simulink model "WSCC_Indian_400kV"  (R2022a)
settings: Solver=FixedStepDiscrete  StartTime=0.0  StopTime=1  FixedStep=5e-7  RelTol=1e-3
PreLoadFcn:
  | tf=1e-3
  | to=20e-3
model workspace (MAT data in the model file):
  tf = 0.001
  to = 0.02
undefined symbols (not defined in the file or in its folder): D1, Delta
libraries: spsFourierLib x72, spsThreePhaseVIMeasurementLib x21, spsThreePhaseBreakerLib x12, spsDistributedParametersLineLib x12, spsLoadFlowBusLib x9, spsThreePhaseParallelRLCLoadLib x6, spsThreePhaseSeriesRLCLoadLib x3, spsThreePhaseSourceLib x3, spsThreePhaseTransformerTwoWindingsLib x3, spsThreePhaseFaultLib x1, spspowerguiLib x1
(part 1 of 2)
settings Model: ParameterArgumentNames=tf,to  Creator=MARI  LastModifiedBy=Dell
settings SolverCC: AlgebraicLoopSolver=TrustRegion
settings DataIOCC: SignalLogging=off  DSMLogging=off
settings DebuggingCC: SFMachineParentedDataDiag=warning  ArithmeticOperatorsInVariantConditions=warning
settings SFSimCC: SimUseLocalCustomCode=off  CustomCodeUndefinedFunction=UseInterfaceOnly
settings RTWCC: RTWUseLocalCustomCode=off  DLArmComputeVersion=19.05

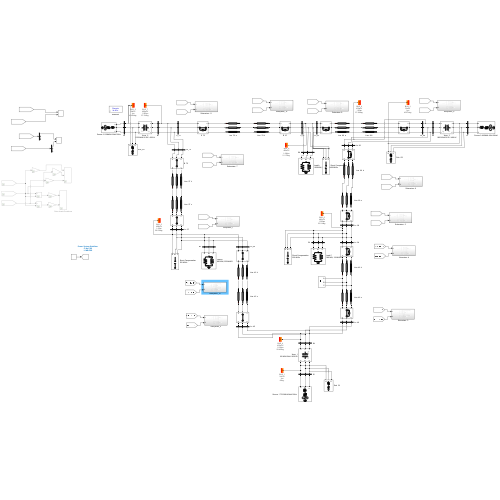
[thumbnail: Simulink's stored preview of the top-level diagram]
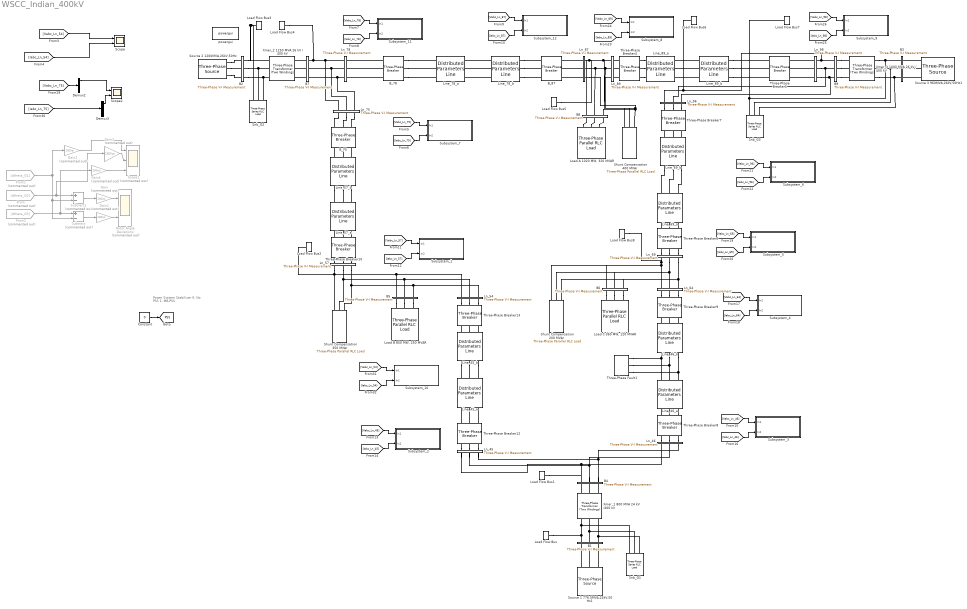
== system WSCC_Indian_400kV ==
  note: Power System Stabilizer
      | 0: No PSS
      | 1: MB-PSS
  B1 : spsThreePhaseVIMeasurementLib/Three-Phase V-I Measurement  VoltageMeasurement=phase-to-ground  SetLabelV=on  LabelV=Vabc_G1  Vpu=off  VpuLL=off  CurrentMeasurement=yes  SetLabelI=on  LabelI=Iabc_G1  Ipu=off  Pbase=100e6  Vbase=500e3  OutputType=Complex  PhasorSimulation=off  PSBequivalent=0
  B2 : spsThreePhaseVIMeasurementLib/Three-Phase V-I Measurement  VoltageMeasurement=phase-to-ground  SetLabelV=on  LabelV=Vabc_G2  Vpu=off  VpuLL=off  CurrentMeasurement=yes  SetLabelI=on  LabelI=Iabc_G2  Ipu=off  Pbase=100e6  Vbase=500e3  OutputType=Complex  PhasorSimulation=off  PSBequivalent=0
  B3 : spsThreePhaseVIMeasurementLib/Three-Phase V-I Measurement  VoltageMeasurement=phase-to-ground  SetLabelV=on  LabelV=Vabc_G3  Vpu=off  VpuLL=off  CurrentMeasurement=yes  SetLabelI=on  LabelI=Iabc_G3  Ipu=off  Pbase=100e6  Vbase=500e3  OutputType=Complex  PhasorSimulation=off  PSBequivalent=0
  B4 : spsThreePhaseVIMeasurementLib/Three-Phase V-I Measurement  VoltageMeasurement=phase-to-ground  SetLabelV=on  LabelV=Vabc_X1  Vpu=off  VpuLL=off  CurrentMeasurement=yes  SetLabelI=on  LabelI=Iabc_X1  Ipu=off  Pbase=100e6  Vbase=500e3  OutputType=Complex  PhasorSimulation=off  PSBequivalent=0
  B5 : spsThreePhaseVIMeasurementLib/Three-Phase V-I Measurement  VoltageMeasurement=phase-to-ground  SetLabelV=on  LabelV=Vabc_Ld_B  Vpu=off  VpuLL=off  CurrentMeasurement=yes  SetLabelI=on  LabelI=Iabc_Ld_B  Ipu=off  Pbase=100e6  Vbase=500e3  OutputType=Complex  PhasorSimulation=off  PSBequivalent=0
  B6 : spsThreePhaseVIMeasurementLib/Three-Phase V-I Measurement  VoltageMeasurement=phase-to-ground  SetLabelV=on  LabelV=Vabc_Ld_C  Vpu=off  VpuLL=off  CurrentMeasurement=yes  SetLabelI=on  LabelI=Iabc_Ld_C  Ipu=off  Pbase=100e6  Vbase=500e3  OutputType=Complex  PhasorSimulation=off  PSBequivalent=0
  B7 : spsThreePhaseVIMeasurementLib/Three-Phase V-I Measurement  VoltageMeasurement=phase-to-ground  SetLabelV=on  LabelV=Vabc_X2  Vpu=off  VpuLL=off  CurrentMeasurement=yes  SetLabelI=on  LabelI=Iabc_X2  Ipu=off  Pbase=100e6  Vbase=500e3  OutputType=Complex  PhasorSimulation=off  PSBequivalent=0
  B8 : spsThreePhaseVIMeasurementLib/Three-Phase V-I Measurement  VoltageMeasurement=phase-to-ground  SetLabelV=on  LabelV=Vabc_Ld_A  Vpu=off  VpuLL=off  CurrentMeasurement=yes  SetLabelI=on  LabelI=Iabc_Ld_A  Ipu=off  Pbase=100e6  Vbase=500e3  OutputType=Complex  PhasorSimulation=off  PSBequivalent=0
  B9 : spsThreePhaseVIMeasurementLib/Three-Phase V-I Measurement  VoltageMeasurement=phase-to-ground  SetLabelV=on  LabelV=Vabc_X3  Vpu=off  VpuLL=off  CurrentMeasurement=yes  SetLabelI=on  LabelI=Iabc_X3  Ipu=off  Pbase=100e6  Vbase=500e3  OutputType=Complex  PhasorSimulation=off  PSBequivalent=0
  B_75 : spsThreePhaseBreakerLib/Three-Phase Breaker  InitialState=closed  SwitchA=on  SwitchB=on  SwitchC=on  SwitchTimes=[500 501]  External=off  BreakerResistance=0.01  SnubberResistance=inf  SnubberCapacitance=inf  Measurements=None
  B_78 : spsThreePhaseBreakerLib/Three-Phase Breaker  InitialState=closed  SwitchA=on  SwitchB=on  SwitchC=on  SwitchTimes=[500 501]  External=off  BreakerResistance=0.01  SnubberResistance=10e6  SnubberCapacitance=inf  Measurements=None
  B_87 : spsThreePhaseBreakerLib/Three-Phase Breaker  InitialState=closed  SwitchA=on  SwitchB=on  SwitchC=on  SwitchTimes=[500 501]  External=off  BreakerResistance=0.01  SnubberResistance=10e6  SnubberCapacitance=inf  Measurements=None
  Constant : Constant  Value=0
  Demux2 : Demux  Outputs=3
  Demux3 : Demux  Outputs=3
  From : From  Commented=on  GotoTag=dtheta_G2
  From1 : From  Commented=on  GotoTag=dtheta_G1
  From2 : From  Commented=on  GotoTag=dtheta_G3
  Gain{,1..4} (5 alike) : Gain  Commented=on  Gain=180/pi
  Line_45_a : spsDistributedParametersLineLib/Distributed Parameters Line  Phases=3  Length=90  Frequency=50  Resistance=[0.0298 0.1619]  Inductance=[1.0568e-03 3.9470e-03]  Capacitance=[11.0414e-09 7.1301e-09]  x1=[-0.00048 -0.000500323391905853 302835.955606375 -284216.33245044;-0.00046 -0.000500693757200361 304615.750015299 -282307.960357671;-0.00044 -0.00050104435596266 306383.518715997 -280388.443230016;-0.00042 -0.00050137517435171 308139.19191999 -278457.856846725;-0.0004 -0.000501686199307369 309882.700316304 -276516.277424041;-0.00038 -0.000501977418550903 311613.975074215 -274563.781612196;-0.00036 -0.000502248820585476 313332.947845957 -272600.446492382;-0.00034 -0.000502500394696601 315039.550769431 -270626.349573707;-0.00032 -0.000502732130952561 316733.716470874 -268641.568790137;-0.0003 -0.000502944020204806 318415.378067527 -266646.18249742;-0.00028 -0.000503136054088312 320084.469170267 -264640.269469989;-0.00026 -0.000503308225021909 321740.923886237 -262623.908897855;-0.00024 -0.000503460526208584 323384.676821441 -260597.180383483;-0.00022 -0.000503592951635747 325015.663083327 -258560.163938643;-0.0002 -0.000503705496075468 326633.818283351 -256512.939981257;-0.00018 -0.000503798155084687 328239.078539515 -254455.589332221;-0.00016 -0.000503870925005383 329831.380478894 -252388.193212216;-0.00014 -0.000503923802964725 331410.661240133 -250310.8332385;-0.00012 -0.000503956786875182 332976.858475933 -248223.591421689;-0.0001 -0.000503969875434606 334529.910355508 -246126.550162516;-8e-05 -0.000503963068126281 336069.755567029 -244019.792248578;-6e-05 -0.000503936365218951 337596.333320043 -241903.400851071;-4e-05 -0.000503889767766798 339109.583347876 -239777.459521504;-2e-05 -0.000503823277609412 340609.445910006 -237642.052188399]  x2=[-0.00048 -0.000256541905604458 288659.111644199 -303840.350628517;-0.00046 -0.000258441737311412 290562.486422962 -302020.666326207;-0.00044 -0.0002603313661811 292454.390292283 -300189.058765133;-0.00042 -0.000262210717614209 294334.748563038 -298345.600254026;-0.0004 -0.000264079717417164 296203.487001901 -296490.363569469;-0.00038 -0.000265938291805053 298060.53183428 -294623.421953032;-0.00036 -0.00026778636740454 299905.809747222 -292744.849108372;-0.00034 -0.000269623871256766 301739.247892317 -290854.719198329;-0.00032 -0.000271450730820224 303560.773888566 -288953.106841995;-0.0003 -0.000273266873973628 305370.315825241 -287040.087111769;-0.00028 -0.000275072229018755 307167.802264724 -285115.735530396;-0.00026 -0.00027686672468328 308953.16224533 -283180.128067981;-0.00024 -0.000278650290123586 310726.325284103 -281233.341138991;-0.00022 -0.000280422854927563 312487.221379602 -279275.451599242;-0.0002 -0.000282184349117389 314235.781014665 -277306.53674286;-0.00018 -0.000283934703152289 315971.935159152 -275326.674299232;-0.00016 -0.000285673847931282 317695.615272669 -273335.942429938;-0.00014 -0.000287401714795911 319406.753307277 -271334.419725662;-0.00012 -0.00028911823553295 321105.281710177 -269322.185203095;-0.0001 -0.0002908233423771 322791.133426374 -267299.318301809;-8e-05 -0.000292516968013663 324464.241901332 -265265.898881127;-6e-05 -0.000294199045581198 326124.54108359 -263222.007216964;-4e-05 -0.000295869508674162 327771.965427381 -261167.723998665;-2e-05 -0.000297528291345534 329406.449895213 -259103.130325814]  x3=[-0.00048 1.74609434734278e-06 236.557476392391 -548.665991316306;-0.00046 1.75692178428303e-06 240.00015435941 -547.16883645487;-0.00044 1.76767986095957e-06 243.433357531282 -545.650080304675;-0.00042 1.77836815266196e-06 246.856950371023 -544.109782823612;-0.0004 1.78898623743472e-06 250.27079772105 -542.548004819988;-0.00038 1.79953369609407e-06 253.674764808515 -540.964807950125;-0.00036 1.8100101122444e-06 257.068717250626 -539.360254715924;-0.00034 1.82041507229472e-06 260.452521059953 -537.7344084624;-0.00032 1.83074816547504e-06 263.826042649714 -536.087333375178;-0.0003 1.84100898385253e-06 267.189148839054 -534.419094477964;-0.00028 1.85119712234765e-06 270.541706858299 -532.729757629971;-0.00026 1.86131217875014e-06 273.883584354198 -531.019389523326;-0.00024 1.87135375373489e-06 277.214649395152 -529.288057680434;-0.00022 1.88132145087771e-06 280.534770476414 -527.535830451311;-0.0002 1.89121487667099e-06 283.843816525291 -525.762777010888;-0.00018 1.90103364053922e-06 287.141656906309 -523.968967356279;-0.00016 1.9107773548544e-06 290.428161426379 -522.154472304017;-0.00014 1.9204456349514e-06 293.703200339928 -520.319363487259;-0.00012 1.93003809914305e-06 296.966644354027 -518.463713352961;-0.0001 1.93955436873531e-06 300.218364633496 -516.587595159012;-8e-05 1.94899406804214e-06 303.458232805986 -514.691082971346;-6e-05 1.95835682440037e-06 306.686120967048 -512.774251661016;-4e-05 1.96764226818442e-06 309.901901685185 -510.837176901241;-2e-05 1.97685003282087e-06 313.105448006881 -508.879935164415]  x4=[-0.00048 -2.71213831700393e-06 1571.48762055538 -1431.8045403172;-0.00046 -2.72644875026853e-06 1580.45283477776 -1421.90239475558;-0.00044 -2.7406515480049e-06 1589.35565542839 -1411.9441149221;-0.00042 -2.75474614951091e-06 1598.19573103915 -1401.93009395259;-0.0004 -2.76873199835581e-06 1606.97271261901 -1391.86072718347;-0.00038 -2.78260854240224e-06 1615.68625366775 -1381.73641213608;-0.00036 -2.79637523382801e-06 1624.33601018969 -1371.55754850106;-0.00034 -2.81003152914771e-06 1632.92164070726 -1361.3245381225;-0.00032 -2.82357688923419e-06 1641.44280627446 -1351.03778498214;-0.0003 -2.83701077933981e-06 1649.89917049027 -1340.69769518337;-0.00028 -2.85033266911761e-06 1658.29039951191 -1330.30467693524;-0.00026 -2.86354203264218e-06 1666.61616206803 -1319.85914053631;-0.00024 -2.87663834843047e-06 1674.87612947177 -1309.36149835848;-0.00022 -2.88962109946236e-06 1683.06997563377 -1298.81216483067;-0.0002 -2.90248977320107e-06 1691.19737707501 -1288.21155642252;-0.00018 -2.91524386161339e-06 1699.25801293959 -1277.56009162789;-0.00016 -2.92788286118975e-06 1707.25156500742 -1266.85819094838;-0.00014 -2.94040627296409e-06 1715.17771770674 -1256.1062768767;-0.00012 -2.95281360253355e-06 1723.03615812663 -1245.30477388001;-0.0001 -2.96510436007801e-06 1730.8265760293 -1234.45410838315;-8e-05 -2.97727806037941e-06 1738.5486638624 -1223.55470875181;-6e-05 -2.9893342228409e-06 1746.20211677112 -1212.60700527563;-4e-05 -3.00127237150584e-06 1753.78663261025 -1201.6114301512;-2e-05 -3.01309203507655e-06 1761.30191195609 -1190.568417465]  x5=0.00047744558650175  V1=[1.62e-10 4.153e+05 4.153e+05;314.2 314.2 314.2;-0.6943 0.8874 -0.6834]  V2=[8.471e-10 4.186e+05 4.186e+05;314.2 314.2 314.2;-0.039 0.8395 -0.7313]  I1=[7.601e-12 598 598;314.2 314.2 314.2;-1.312 0.4775 -1.093]  I2=[4.421e-12 2129 2129;314.2 314.2 314.2;2.105 0.9183 -0.6525]  nHarmo=1  Measurements=None  Decoupling=off  VsMag0=0  VrMag0=0  VsAngle0=0  VrAngle0=0  IsMag0=0  IrMag0=0  IsAngle0=0  IrAngle0=0
      settings: SourceProductBaseCode=PS
  Line_45_b : spsDistributedParametersLineLib/Distributed Parameters Line  Phases=3  Length=60  Frequency=50  Resistance=[0.0298 0.1619]  Inductance=[1.0568e-03 3.9470e-03]  Capacitance=[11.0414e-09 7.1301e-09]  x1=[-0.00032 -0.000271450732280679 303560.773888566 -288953.106841995;-0.0003 -0.000273266875343084 305370.315825241 -287040.087111769;-0.00028 -0.000275072230297158 307167.802264724 -285115.735530396;-0.00026 -0.000276866725870579 308953.16224533 -283180.128067981;-0.00024 -0.000278650291219735 310726.325284103 -281233.341138991;-0.00022 -0.000280422855932519 312487.221379602 -279275.451599242;-0.0002 -0.000282184350031111 314235.781014665 -277306.53674286;-0.00018 -0.000283934703974742 315971.935159152 -275326.674299232;-0.00016 -0.000285673848662433 317695.615272669 -273335.942429938;-0.00014 -0.000287401715435731 319406.753307277 -271334.419725662;-0.00012 -0.000289118236081415 321105.281710177 -269322.185203095;-0.0001 -0.000290823342834187 322791.133426374 -267299.318301809;-8e-05 -0.000292516968379354 324464.241901332 -265265.898881127;-6e-05 -0.000294199045855478 326124.54108359 -263222.007216964;-4e-05 -0.000295869508857022 327771.965427381 -261167.723998665;-2e-05 -0.000297528291436966 329406.449895213 -259103.130325814]  x2=[-0.00032 -0.000113963482428579 293331.273337558 -300866.465593188;-0.0003 -0.000116825548862926 295215.870543759 -299017.484128223;-0.00028 -0.000119683003224641 297088.813132882 -297156.697964984;-0.00026 -0.000122535732706319 298950.02716436 -295284.180564123;-0.00024 -0.000125383624687085 300799.43916065 -293400.005849421;-0.00022 -0.000128226566737039 302636.976110133 -291504.24820487;-0.0002 -0.000131064446621698 304462.565469997 -289596.982471735;-0.00018 -0.000133897152306422 306276.1351691 -287678.283945601;-0.00016 -0.000136724571960841 308077.613610815 -285748.228373401;-0.00014 -0.00013954659396327 309866.929675857 -283806.891950424;-0.00012 -0.000142363106905111 311644.012725094 -281854.351317308;-0.0001 -0.000145173999595256 313408.792602328 -279890.683557014;-8e-05 -0.000147979161064475 315161.199637071 -277915.966191783;-6e-05 -0.000150778480569796 316901.164647296 -275930.277180075;-4e-05 -0.000153571847598878 318628.618942162 -273933.694913492;-2e-05 -0.000156359151874374 320343.494324732 -271926.298213684]  x3=[-0.00032 2.11081364469373e-06 309.410896766023 -506.244452632187;-0.0003 2.11946097416425e-06 312.58559603185 -504.290386606476;-0.00028 2.12802463094461e-06 315.747954953577 -502.316412059784;-0.00026 2.13650427695629e-06 318.89784868669 -500.322606921248;-0.00024 2.14489957743741e-06 322.035152878777 -498.30904990288;-0.00022 2.15321020095586e-06 325.159743674441 -496.275820496463;-0.0002 2.16143581942247e-06 328.271497720188 -494.222998970414;-0.00018 2.1695761081039e-06 331.370292169295 -492.15066636661;-0.00016 2.17763074563549e-06 334.456004686665 -490.058904497196;-0.00014 2.18559941403394e-06 337.528513453649 -487.947795941347;-0.00012 2.19348179870987e-06 340.587697172864 -485.817424042015;-0.0001 2.20127758848023e-06 343.633435072975 -483.667872902634;-8e-05 2.20898647558059e-06 346.665606913463 -481.499227383803;-6e-05 2.21660815567728e-06 349.684092989376 -479.311573099934;-4e-05 2.22414232787943e-06 352.688774136054 -477.104996415872;-2e-05 2.23158869475082e-06 355.679531733829 -474.879584443485]  x4=[-0.00032 -2.57395052999193e-06 1550.37311665751 -1453.95656083358;-0.0003 -2.58898708897482e-06 1559.47793199607 -1444.18664347805;-0.00028 -2.60392143918049e-06 1568.52118181613 -1434.35971210668;-0.00026 -2.61875299102637e-06 1577.50250910567 -1424.4761546699;-0.00024 -2.63348115898819e-06 1586.42155929727 -1414.53636135362;-0.00022 -2.64810536162309e-06 1595.27798028209 -1404.54072456387;-0.0002 -2.66262502159259e-06 1604.07142242381 -1394.48963891127;-0.00018 -2.67703956568539e-06 1612.80153857238 -1384.38350119548;-0.00016 -2.69134842483997e-06 1621.46798407777 -1374.22271038951;-0.00014 -2.70555103416705e-06 1630.07041680354 -1364.00766762397;-0.00012 -2.71964683297195e-06 1638.60849714038 -1353.73877617127;-0.0001 -2.73363526477667e-06 1647.08188801951 -1343.41644142966;-8e-05 -2.74751577734187e-06 1655.49025492595 -1333.04107090725;-6e-05 -2.76128782268868e-06 1663.83326591178 -1322.61307420588;-4e-05 -2.77495085712033e-06 1672.11059160921 -1312.13286300502;-2e-05 -2.78850434124362e-06 1680.3219052436 -1301.60085104546]  x5=0.000318297057667833  V1=[8.377e-10 4.186e+05 4.186e+05;314.2 314.2 314.2;-0.02057 0.8395 -0.7313]  V2=[8.866e-10 4.202e+05 4.202e+05;314.2 314.2 314.2;-0.5299 0.7927 -0.7781]  I1=[5.663e-12 593.1 593.1;314.2 314.2 314.2;-2.774 0.5529 -1.018]  I2=[8.582e-12 2124 2124;314.2 314.2 314.2;-0.07241 0.8375 -0.7333]  nHarmo=1  Measurements=None  Decoupling=off  VsMag0=0  VrMag0=0  VsAngle0=0  VrAngle0=0  IsMag0=0  IrMag0=0  IsAngle0=0  IrAngle0=0
      settings: SourceProductBaseCode=PS
  Line_46_a : spsDistributedParametersLineLib/Distributed Parameters Line  Phases=3  Length=60  Frequency=50  Resistance=[0.0298 0.1619]  Inductance=[1.0568e-03 3.9470e-03]  Capacitance=[11.0414e-09 7.1301e-09]  x1=[-0.00032 -0.000503298405632093 316737.218945027 -268645.514115454;-0.0003 -0.000503514299837074 318418.905261583 -266650.105738309;-0.00028 -0.000503710316159651 320088.02094498 -264644.170471566;-0.00026 -0.000503886446861437 321744.500101388 -262627.787506117;-0.00024 -0.000504042684989092 323388.277335847 -260601.036445308;-0.00022 -0.000504179024374603 325019.287754846 -258563.997301801;-0.0002 -0.000504295459635525 326637.466968887 -256516.750494413;-0.00018 -0.000504391986175192 328242.751095025 -254459.376844942;-0.00016 -0.000504468600182903 329835.076759391 -252391.957574977;-0.00014 -0.000504525298634067 331414.381099695 -250314.574302692;-0.00012 -0.000504562079290327 332980.601767706 -248227.30903962;-0.0001 -0.000504578940699645 334533.676931713 -246130.244187421;-8e-05 -0.000504575882196361 336073.545278968 -244023.462534624;-6e-05 -0.000504552903901221 337600.146018105 -241907.047253361;-4e-05 -0.000504510006721368 339113.418881542 -239781.081896084;-2e-05 -0.000504447192350309 340613.304127856 -237645.650392264]  x2=[-0.00032 -0.000448622268654471 316728.936456653 -276237.738045629;-0.0003 -0.000449366397899025 318458.325972699 -274242.231844579;-0.00028 -0.000450092786927629 320175.143299322 -272235.899029795;-0.00026 -0.000450801407063687 321879.320659516 -270218.818807859;-0.00024 -0.000451492230332091 323570.790775277 -268191.070809645;-0.00022 -0.000452165229460319 325249.486870259 -266152.735087172;-0.0002 -0.000452820377879519 326915.342672416 -264103.892110445;-0.00018 -0.000453457649725553 328568.292416613 -262044.622764275;-0.00016 -0.000454077019840019 330208.270847224 -259975.008345091;-0.00014 -0.000454678463771247 331835.21322071 -257895.130557726;-0.00012 -0.000455261957775259 333449.05530817 -255805.071512194;-0.0001 -0.000455827478816712 335049.733397883 -253704.913720447;-8e-05 -0.000456375004569803 336637.184297819 -251594.740093119;-6e-05 -0.000456904513419152 338211.345338134 -249474.633936251;-4e-05 -0.000457415984460657 339772.154373645 -247344.678948004;-2e-05 -0.000457909397502318 341319.549786285 -245204.959215354]  x3=[-0.00032 5.29696817540032e-07 614.190534101928 -930.892484413467;-0.0003 5.32789423649159e-07 620.027341995361 -927.015061847602;-0.00028 5.35860996144122e-07 625.839672270988 -923.101042314399;-0.00026 5.38911413764499e-07 631.627295467964 -919.150580332648;-0.00024 5.41940556085024e-07 637.389983100834 -915.163831859823;-0.00022 5.44948303520346e-07 643.127507668557 -911.140954285927;-0.0002 5.47934537329745e-07 648.839642663489 -907.08210642728;-0.00018 5.50899139621826e-07 654.526162580319 -902.987448520245;-0.00016 5.53841993359164e-07 660.186842924979 -898.857142214903;-0.00014 5.56762982362934e-07 665.821460223501 -894.691350568678;-0.00012 5.59661991317491e-07 671.429792030843 -890.490238039888;-0.0001 5.62538905774926e-07 677.011616939667 -886.253970481265;-8e-05 5.65393612159581e-07 682.566714589084 -881.982715133396;-6e-05 5.68225997772538e-07 688.09486567335 -877.676640618131;-4e-05 5.71035950796061e-07 693.595851950527 -873.335916931917;-2e-05 5.73823360298017e-07 699.069456251095 -868.960715439093]  x4=[-0.00032 -1.78624242588469e-06 1367.9660006306 -888.484145915788;-0.0003 -1.79101262468386e-06 1373.52147194241 -879.871480682929;-0.00028 -1.7957121173713e-06 1379.02271897835 -871.224079630594;-0.00026 -1.80034071841911e-06 1384.46952455861 -862.542284143369;-0.00024 -1.80489824509802e-06 1389.86167365264 -853.826436963676;-0.00022 -1.80938451748471e-06 1395.19895338761 -845.076882178236;-0.0002 -1.8137993584688e-06 1400.48115305686 -836.293965204491;-0.00018 -1.81814259375995e-06 1405.7080641282 -827.478032776965;-0.00016 -1.82241405189465e-06 1410.87948025213 -818.629432933574;-0.00014 -1.82661356424305e-06 1415.99519726999 -809.748515001889;-0.00012 -1.8307409650156e-06 1421.05501322203 -800.835629585343;-0.0001 -1.83479609126959e-06 1426.05872835539 -791.891128549391;-8e-05 -1.83877878291556e-06 1431.00614513196 -782.915365007619;-6e-05 -1.84268888272368e-06 1435.89706823619 -773.908693307803;-4e-05 -1.8465262363299e-06 1440.73130458281 -764.871469017918;-2e-05 -1.85029069224207e-06 1445.50866332446 -755.804048912106]  x5=0.000318297057667833  V1=[2.78e-10 4.153e+05 4.153e+05;314.2 314.2 314.2;2.169 0.8713 -0.6995]  V2=[5.247e-10 4.221e+05 4.221e+05;314.2 314.2 314.2;2.009 0.8508 -0.72]  I1=[2.389e-12 1113 1113;314.2 314.2 314.2;0.1121 0.5869 -0.9839]  I2=[3.387e-12 1627 1627;314.2 314.2 314.2;-2.917 0.9662 -0.6046]  nHarmo=1  Measurements=None  Decoupling=off  VsMag0=0  VrMag0=0  VsAngle0=0  VrAngle0=0  IsMag0=0  IrMag0=0  IsAngle0=0  IrAngle0=0
      settings: SourceProductBaseCode=PS
  Line_46_b : spsDistributedParametersLineLib/Distributed Parameters Line  Phases=3  Length=60  Frequency=50  Resistance=[0.0298 0.1619]  Inductance=[1.0568e-03 3.9470e-03]  Capacitance=[11.0414e-09 7.1301e-09]  x1=[-0.00032 -0.0004486222534458 316728.936456653 -276237.738045629;-0.0003 -0.000449366382726964 318458.325972699 -274242.231844579;-0.00028 -0.000450092771792776 320175.143299322 -272235.899029795;-0.00026 -0.00045080139196664 321879.320659516 -270218.818807859;-0.00024 -0.000451492215273444 323570.790775277 -268191.070809645;-0.00022 -0.000452165214440668 325249.486870259 -266152.735087172;-0.0002 -0.000452820362899457 326915.342672416 -264103.892110445;-0.00018 -0.000453457634785671 328568.292416613 -262044.622764275;-0.00016 -0.000454077004940908 330208.270847224 -259975.008345091;-0.00014 -0.000454678448913494 331835.21322071 -257895.130557726;-0.00012 -0.000455261942959451 333449.05530817 -255805.071512194;-0.0001 -0.000455827464043434 335049.733397883 -253704.913720447;-8e-05 -0.000456374989839637 336637.184297819 -251594.740093119;-6e-05 -0.000456904498732681 338211.345338134 -249474.633936251;-4e-05 -0.000457415969818461 339772.154373645 -247344.678948004;-2e-05 -0.000457909382904974 341319.549786285 -245204.959215354]  x2=[-0.00032 -0.00038962046774844 315510.702102501 -282567.317791598;-0.0003 -0.000390881722330777 317279.885326274 -280579.340991918;-0.00028 -0.000392127545572012 319036.542883445 -278580.287400285;-0.00026 -0.000393357888289179 320780.60542418 -276570.235935911;-0.00024 -0.000394572701910452 322512.004095878 -274549.265952186;-0.00022 -0.00039577193847707 324230.670545883 -272517.457233545;-0.0002 -0.000396955550645228 325936.536924187 -270474.889992317;-0.00018 -0.000398123491687943 327629.535886105 -268421.644865559;-0.00016 -0.000399275715496902 329309.600594939 -266357.802911874;-0.00014 -0.000400412176584284 330976.664724609 -264283.445608207;-0.00012 -0.000401532830084549 332630.662462279 -262198.654846633;-0.0001 -0.000402637631756217 334271.52851095 -260103.512931123;-8e-05 -0.000403726537983609 335899.19809204 -257998.10257429;-6e-05 -0.000404799505778572 337513.606947941 -255882.50689413;-4e-05 -0.000405856492782175 339114.691344555 -253756.80941074;-2e-05 -0.00040689745726638 340702.388073812 -251621.094043016]  x3=[-0.00032 5.92049821364135e-07 670.724909582166 -889.576841853896;-0.0003 5.94839162960827e-07 676.301009405037 -885.345021202816;-0.00028 5.97605021325893e-07 681.85041002207 -881.078248646252;-0.00026 6.00347287267981e-07 687.37289235243 -876.776692629079;-0.00024 6.03065852527127e-07 692.868238377971 -872.440522969363;-0.00022 6.05760609779029e-07 698.336231151841 -868.069910851658;-0.0002 6.08431452639286e-07 703.776654807049 -863.665028820247;-0.00018 6.11078275667593e-07 709.189294564983 -859.226050772328;-0.00016 6.13700974371911e-07 714.573936743895 -854.753151951156;-0.00014 6.16299445212586e-07 719.93036876733 -850.246508939117;-0.00012 6.18873585606436e-07 725.258379172525 -845.70629965076;-0.0001 6.21423293930809e-07 730.557757618751 -841.132703325774;-8e-05 6.23948469527584e-07 735.828294895622 -836.525900521911;-6e-05 6.26449012707153e-07 741.06978293135 -831.886073107856;-4e-05 6.28924824752353e-07 746.282014800962 -827.213404256053;-2e-05 6.31375807922364e-07 751.46478473447 -822.508078435466]  x4=[-0.00032 -1.68620528731294e-06 1306.03920719579 -974.477686481741;-0.0003 -1.69201605091698e-06 1312.13621068535 -966.252418769138;-0.00028 -1.69776001662452e-06 1318.18141328405 -957.989005065531;-0.00026 -1.70343695767363e-06 1324.17457633764 -949.687771596344;-0.00024 -1.70904664994841e-06 1330.1154632463 -941.34904608006;-0.00022 -1.7145888719878e-06 1336.003839474 -932.973157715285;-0.0002 -1.72006340499437e-06 1341.83947255773 -924.560437167749;-0.00018 -1.72547003284294e-06 1347.62213211667 -916.111216557255;-0.00016 -1.73080854208908e-06 1353.35158986133 -907.625829444565;-0.00014 -1.73607872197761e-06 1359.02761960254 -899.104610818232;-0.00012 -1.74128036445083e-06 1364.64999726035 -890.547897081379;-0.0001 -1.74641326415681e-06 1370.21850087293 -881.95602603841;-8e-05 -1.75147721845747e-06 1375.73291060528 -873.329336881685;-6e-05 -1.75647202743654e-06 1381.19300875795 -864.668170178118;-4e-05 -1.76139749390754e-06 1386.59857977562 -855.972867855742;-2e-05 -1.76625342342147e-06 1391.9494102556 -847.243773190203]  x5=0.000318297057667833  V1=[5.267e-10 4.221e+05 4.221e+05;314.2 314.2 314.2;2.115 0.9152 -0.6556]  V2=[4.511e-10 4.235e+05 4.235e+05;314.2 314.2 314.2;1.521 0.9087 -0.6621]  I1=[7.622e-12 1116 1116;314.2 314.2 314.2;-1.047 0.7461 -0.8247]  I2=[9.859e-12 1633 1633;314.2 314.2 314.2;1.521 0.998 -0.5728]  nHarmo=1  Measurements=None  Decoupling=off  VsMag0=0  VrMag0=0  VsAngle0=0  VrAngle0=0  IsMag0=0  IrMag0=0  IsAngle0=0  IrAngle0=0
      settings: SourceProductBaseCode=PS
  Line_57_a : spsDistributedParametersLineLib/Distributed Parameters Line  Phases=3  Length=30  Frequency=50  Resistance=[0.0298 0.1619]  Inductance=[1.0568e-03 3.9470e-03]  Capacitance=[11.0414e-09 7.1301e-09]  x1=[-0.00016 -0.000136685335636007 0 0;-0.00014 -0.000139507274512133 0 0;-0.00012 -0.000142323705879936 311649.319809917 -281855.585865267;-0.0001 -0.000145134518551528 313414.107339236 -279891.884735427;-8e-05 -0.000147939601560837 315166.521816248 -277917.133953229;-6e-05 -0.00015073884416799 316906.494058631 -275931.411478452;-4e-05 -0.000153532135863682 318633.955375258 -273934.795704021;-2e-05 -0.000156319366373539 320348.837568917 -271927.365452907]  x2=[-0.00016 -0.000142334759161942 0 0;-0.00014 -0.000145485701567132 0 0;-0.00012 -0.000148630900445936 318234.901438311 -270572.485792383;-0.0001 -0.000151770231631287 319928.665631613 -268567.629223678;-8e-05 -0.000154903571187765 321609.799589001 -266552.170064833;-6e-05 -0.00015803079541649 323278.236942185 -264526.187882724;-4e-05 -0.000161151780860005 324933.911824116 -262489.762659659;-2e-05 -0.000164266404307147 326576.758871584 -260442.974790219]  x3=[-0.00016 1.19338307706653e-06 0 0;-0.00014 1.18748533428075e-06 0 0;-0.00012 1.18154071160727e-06 2171.66221780702 -1479.63246739289;-0.0001 1.17554944372961e-06 2180.91609483756 -1465.95839437254;-8e-05 1.16951176717279e-06 2190.083873035 -1452.22644782491;-6e-05 1.16342792029392e-06 2199.16519047116 -1438.43716986372;-4e-05 1.15729814327286e-06 2208.15968863118 -1424.59110486607;-2e-05 1.15112267810272e-06 2217.06701242766 -1410.68879945089]  x4=[-0.00016 -1.53469559491092e-06 0 0;-0.00014 -1.53684582012509e-06 0 0;-0.00012 -1.53893537329777e-06 -168.780868301187 -334.860878995869;-0.0001 -1.540964171937e-06 -166.673557597244 -335.914743614145;-8e-05 -1.54293213594927e-06 -164.559666906638 -336.955346893522;-6e-05 -1.54483918764273e-06 -162.439279682154 -337.982647752763;-4e-05 -1.54668525173026e-06 -160.312479633049 -338.99660563579;-2e-05 -1.5484702553324e-06 -158.179350721746 -339.997180513281]  x5=0.000159148528833917  V1=[8.847e-10 4.202e+05 4.202e+05;314.2 314.2 314.2;0.04885 0.841 -0.7298]  V2=[4.139e-10 4.177e+05 4.177e+05;314.2 314.2 314.2;-0.2267 0.8716 -0.6992]  I1=[1.496e-11 2628 2628;314.2 314.2 314.2;1.536 0.9781 -0.5927]  I2=[1.402e-11 375 375;314.2 314.2 314.2;-1.159 -0.4607 -2.031]  nHarmo=1  Measurements=None  Decoupling=off  VsMag0=0  VrMag0=0  VsAngle0=0  VrAngle0=0  IsMag0=0  IrMag0=0  IsAngle0=0  IrAngle0=0
      settings: SourceProductBaseCode=PS
  Line_57_b : spsDistributedParametersLineLib/Distributed Parameters Line  Phases=3  Length=90  Frequency=50  Resistance=[0.0298 0.1619]  Inductance=[1.0568e-03 3.9470e-03]  Capacitance=[11.0414e-09 7.1301e-09]  x1=[-0.00048 -9.12407184270517e-05 285665.964942323 -304758.722695604;-0.00046 -9.44665005766934e-05 287575.1690668 -302957.826637054;-0.00044 -9.76885533506449e-05 289473.02021601 -301144.970322255;-0.00042 -0.00010090674954778 291359.443466039 -299320.225319671;-0.0004 -0.000104120962119222 293234.364344127 -297483.663667109;-0.00038 -0.000107331064173364 295097.708831609 -295635.357868879;-0.00036 -0.000110536928980873 296949.403366834 -293775.38089293;-0.00034 -0.000113738429979695 298789.374848073 -291903.806167966;-0.00032 -0.000116935440780052 300617.550636403 -290020.707580555;-0.0003 -0.000120127835169433 302433.858558572 -288126.159472203;-0.00028 -0.000123315487117574 304238.226909856 -286220.236636427;-0.00026 -0.000126498270781433 306030.584456881 -284303.014315795;-0.00024 -0.000129676060510161 307810.860440439 -282374.568198963;-0.00022 -0.000132848730850062 309578.984578284 -280434.974417682;-0.0002 -0.000136016156549542 311334.887067902 -278484.309543791;-0.00018 -0.000139178212564058 313078.49858927 -276522.650586202;-0.00016 -0.000142334774061053 314809.750307589 -274550.07498785;-0.00014 -0.000145485716424885 316528.573876007 -272566.660622643;-0.00012 -0.000148630915261744 318234.901438311 -270572.485792383;-0.0001 -0.000151770246404565 319928.665631613 -268567.629223678;-8e-05 -0.00015490358591793 321609.799589001 -266552.170064833;-6e-05 -0.000158030810102961 323278.236942185 -264526.187882724;-4e-05 -0.000161151795502201 324933.911824116 -262489.762659659;-2e-05 -0.00016426641890449 326576.758871584 -260442.974790219]  x2=[-0.00048 -9.20501105598107e-05 307474.245287704 -271342.543354409;-0.00046 -9.62161844147352e-05 309173.060269381 -269405.282337222;-0.00044 -0.000100378459819447 310859.669628028 -267457.385660785;-0.00042 -0.000104536772454441 312534.006779195 -265498.930224722;-0.0004 -0.000108690958156655 314196.005622918 -263529.993345501;-0.00038 -0.000112840852925948 315845.600546329 -261550.652753379;-0.00036 -0.000116986292931583 317482.726426245 -259560.986589332;-0.00034 -0.000121127114518686 319107.318631739 -257561.073401974;-0.00032 -0.00012526315421471 320719.313026693 -255550.992144453;-0.0003 -0.00012939424873589 322318.645972327 -253530.822171336;-0.00028 -0.000133520234993689 323905.254329717 -251500.643235474;-0.00026 -0.000137640950101234 325479.07546228 -249460.535484855;-0.00024 -0.000141756231379748 327040.047238254 -247410.57945944;-0.00022 -0.000145865916364972 328588.108033145 -245350.856087983;-0.0002 -0.000149969842813581 330123.196732163 -243281.446684835;-0.00018 -0.000154067848709585 331645.252732637 -241202.432946737;-0.00016 -0.000158159772270728 333154.215946399 -239113.89694959;-0.00014 -0.000162245451954875 334650.026802168 -237015.921145221;-0.00012 -0.000166324726466388 336132.626247891 -234908.588358121;-0.0001 -0.000170397434762493 337601.955753081 -232791.981782181;-8e-05 -0.000174463416059641 339057.957311125 -230666.184977403;-6e-05 -0.000178522509839852 340500.573441575 -228531.281866607;-4e-05 -0.000182574555857054 341929.747192416 -226387.35673211;-2e-05 -0.000186619394143409 343345.422142315 -224234.494212407]  x3=[-0.00048 1.24031834139039e-06 2040.99466411098 -1646.04250236012;-0.00046 1.23484713592412e-06 2051.29669861567 -1633.18614760162;-0.00044 1.22932718080732e-06 2061.51775143907 -1620.26531745047;-0.00042 1.22375869395836e-06 2071.65741907154 -1607.28052199893;-0.0004 1.21814189521158e-06 2081.71530121634 -1594.23227386449;-0.00038 1.21247700630856e-06 2091.69100080552 -1581.12108816963;-0.00036 1.20676425088944e-06 2101.58412401554 -1567.94748252153;-0.00034 1.20100385448399e-06 2111.39428028283 -1554.71197699158;-0.00032 1.19519604450282e-06 2121.12108231922 -1541.41509409486;-0.0003 1.18934105022832e-06 2130.76414612722 -1528.05735876956;-0.00028 1.18343910280563e-06 2140.32309101518 -1514.63929835619;-0.00026 1.17749043523354e-06 2149.79753961234 -1501.16144257679;-0.00024 1.17149528235525e-06 2159.18711788367 -1487.62432351405;-0.00022 1.16545388084913e-06 2168.4914551447 -1474.02847559023;-0.0002 1.15936646921937e-06 2177.71018407614 -1460.37443554613;-0.00018 1.15323328778656e-06 2186.84294073835 -1446.66274241988;-0.00016 1.14705457867821e-06 2195.88936458574 -1432.89393752565;-0.00014 1.14083058581915e-06 2204.84909848097 -1419.06856443227;-0.00012 1.13456155492199e-06 2213.72178870911 -1405.18716894179;-0.0001 1.12824773347731e-06 2222.50708499152 -1391.25029906796;-8e-05 1.12188937074399e-06 2231.20464049976 -1377.25850501452;-6e-05 1.1154867177393e-06 2239.81411186923 -1363.21233915354;-4e-05 1.109040027229e-06 2248.33515921273 -1349.11235600361;-2e-05 1.10254955371742e-06 2256.76744613392 -1334.95911220792]  x4=[-0.00048 -1.36536711592803e-06 -225.806854679022 -296.290609394368;-0.00046 -1.36980338852497e-06 -223.94076088962 -297.70353783866;-0.00044 -1.37418558362962e-06 -222.065826302425 -299.10471345703;-0.00042 -1.37851352824041e-06 -220.182124936646 -300.494080933461;-0.0004 -1.38278705149749e-06 -218.289731157586 -301.871585418105;-0.00038 -1.38700598468949e-06 -216.388719673713 -303.237172529444;-0.00036 -1.39117016126016e-06 -214.479165533703 -304.590788356437;-0.00034 -1.39527941681492e-06 -212.561144123485 -305.932379460648;-0.00032 -1.3993335891274e-06 -210.63473116326 -307.261892878358;-0.0003 -1.40333251814583e-06 -208.700002704513 -308.579276122654;-0.00028 -1.40727604599933e-06 -206.757035127012 -309.884477185501;-0.00026 -1.41116401700418e-06 -204.805905135788 -311.177444539796;-0.00024 -1.41499627766994e-06 -202.846689758113 -312.458127141402;-0.00022 -1.41877267670552e-06 -200.879466340455 -313.726474431162;-0.0002 -1.42249306502515e-06 -198.904312545428 -314.982436336898;-0.00018 -1.42615729575427e-06 -196.921306348719 -316.225963275383;-0.00016 -1.42976522423533e-06 -194.93052603602 -317.457006154303;-0.00014 -1.43331670803348e-06 -192.932050199927 -318.675516374194;-0.00012 -1.43681160694223e-06 -190.925957736844 -319.881445830359;-0.0001 -1.44024978298896e-06 -188.912327843868 -321.074746914767;-8e-05 -1.44363110044035e-06 -186.891240015659 -322.255372517935;-6e-05 -1.44695542580779e-06 -184.862774041302 -323.423276030785;-4e-05 -1.45022262785261e-06 -182.827010001162 -324.578411346487;-2e-05 -1.45343257759126e-06 -180.784028263718 -325.720732862276]  x5=0.00047744558650175  V1=[4.309e-10 4.177e+05 4.177e+05;314.2 314.2 314.2;-0.354 0.8072 -0.7636]  V2=[3.73e-10 4.101e+05 4.101e+05;314.2 314.2 314.2;-0.5088 0.9019 -0.6689]  I1=[1.704e-12 2622 2622;314.2 314.2 314.2;-1.588 0.9462 -0.6246]  I2=[3.147e-12 372.5 372.5;314.2 314.2 314.2;-0.7702 -0.5974 -2.168]  nHarmo=1  Measurements=None  Decoupling=off  VsMag0=0  VrMag0=0  VsAngle0=0  VrAngle0=0  IsMag0=0  IrMag0=0  IsAngle0=0  IrAngle0=0
      settings: SourceProductBaseCode=PS
  Line_69_a : spsDistributedParametersLineLib/Distributed Parameters Line  Phases=3  Length=70  Frequency=50  Resistance=[0.0298 0.1619]  Inductance=[1.0568e-03 3.9470e-03]  Capacitance=[11.0414e-09 7.1301e-09]  x1=[-0.00038 -0.000385730585135957 310131.589648991 -288465.723126779;-0.00036 -0.000387037750228063 311937.93958175 -286511.427635631;-0.00034 -0.000388329635732504 313731.974738778 -284545.821163906;-0.00032 -0.000389606190647853 315513.624294639 -282568.981310382;-0.0003 -0.000390867364577909 317282.817912859 -280580.986117312;-0.00028 -0.000392113107733682 319039.485748702 -278581.914067342;-0.00026 -0.000393343370935368 320783.558451931 -276571.844080412;-0.00024 -0.000394558105614281 322514.967169542 -274550.855510646;-0.00022 -0.000395757263814776 324233.643548483 -272519.02814321;-0.0002 -0.00039694079819614 325939.519738354 -270476.44219117;-0.00018 -0.000398108662034464 327632.528394083 -268423.178292322;-0.00016 -0.000399260809224481 329312.602678589 -266359.31750601;-0.00014 -0.000400397194281394 330979.676265413 -264284.941309923;-0.00012 -0.000401517772342667 332633.683341347 -262200.13159688;-0.0001 -0.000402622499169796 334274.558609023 -260104.970671602;-8e-05 -0.000403711331150058 335902.237289494 -257999.541247452;-6e-05 -0.000404784225298231 337516.655124794 -255883.926443179;-4e-05 -0.000405841139258291 339117.748380471 -253758.209779634;-2e-05 -0.000406882031305084 340705.453848105 -251622.475176471]  x2=[-0.00038 -0.000329257561364633 316167.901537245 -274630.335422951;-0.00036 -0.000330626019838311 317887.202585653 -272638.386013764;-0.00034 -0.000331981425762849 319593.953991614 -270635.673307929;-0.00032 -0.000333323725629141 321288.088375503 -268622.276369114;-0.0003 -0.000334652866445486 322969.538855796 -266598.274682783;-0.00028 -0.000335968795739682 324638.239051708 -264563.748153057;-0.00026 -0.000337271461561093 326294.123085812 -262518.77709956;-0.00024 -0.000338560812482702 327937.125586641 -260463.442254247;-0.00022 -0.000339836797603144 329567.181691271 -258397.824758218;-0.0002 -0.00034109936654871 331184.227047877 -256322.006158516;-0.00018 -0.00034234846947534 332788.197818277 -254236.068404905;-0.00016 -0.00034358405707059 334379.030680451 -252140.093846634;-0.00014 -0.000344806080555577 335956.662831044 -250034.165229192;-0.00012 -0.000346014491686906 337521.031987837 -247918.365691034;-0.0001 -0.000347209242758575 339072.076392217 -245792.778760302;-8e-05 -0.000348390286603858 340609.734811604 -243657.488351529;-6e-05 -0.000349557576597165 342133.946541879 -241512.578762325;-4e-05 -0.000350711066655886 343644.651409772 -239358.134670047;-2e-05 -0.00035185071124221 345141.78977524 -237194.241128459]  x3=[-0.00038 -3.05480858220587e-07 1574.64841641218 -1169.47472235691;-0.00036 -3.03500760707191e-07 1581.96531223115 -1159.55789523395;-0.00034 -3.0150868150344e-07 1589.21975476835 -1149.59529075076;-0.00032 -2.99504699253208e-07 1596.41145763082 -1139.58730221392;-0.0003 -2.97488893070284e-07 1603.54013690243 -1129.53432472167;-0.00028 -2.95461342535244e-07 1610.60551115514 -1119.43675514835;-0.00026 -2.93422127692311e-07 1617.60730146006 -1109.29499212873;-0.00024 -2.91371329046197e-07 1624.54523139852 -1099.10943604223;-0.00022 -2.89309027558919e-07 1631.4190270729 -1088.88048899717;-0.0002 -2.8723530464661e-07 1638.22841711753 -1078.60855481487;-0.00018 -2.85150242176299e-07 1644.97313270935 -1068.2940390137;-0.00016 -2.83053922462682e-07 1651.65290757853 -1057.93734879308;-0.00014 -2.80946428264872e-07 1658.26747801901 -1047.53889301741;-0.00012 -2.78827842783132e-07 1664.81658289886 -1037.09908219992;-0.0001 -2.76698249655588e-07 1671.29996367065 -1026.61832848646;-8e-05 -2.74557732954931e-07 1677.71736438159 -1016.09704563924;-6e-05 -2.72406377185096e-07 1684.06853168369 -1005.5356490205;-4e-05 -2.70244267277923e-07 1690.35321484376 -994.934555576088;-2e-05 -2.68071488589811e-07 1696.57116575325 -984.294183819023]  x4=[-0.00038 -6.11227831457646e-07 371.379104799812 -717.271264081693;-0.00036 -6.17113811725719e-07 375.878492705863 -714.923677386024;-0.00034 -6.22975429397174e-07 380.36304157263 -712.547866727717;-0.00032 -6.2881245306538e-07 384.832574357801 -710.143925899709;-0.0003 -6.34624652294639e-07 389.286914611875 -707.711949805468;-0.00028 -6.40411797629277e-07 393.725886485127 -705.252034455246;-0.00026 -6.46173660602706e-07 398.149314734546 -702.764276962288;-0.00024 -6.5191001374644e-07 402.557024730761 -700.248775539001;-0.00022 -6.5762063059908e-07 406.948842464928 -697.705629493073;-0.0002 -6.63305285715251e-07 411.324594555602 -695.134939223557;-0.00018 -6.68963754674502e-07 415.684108255583 -692.536806216901;-0.00016 -6.74595814090169e-07 420.027211458736 -689.911333042949;-0.00014 -6.80201241618188e-07 424.353732706782 -687.258623350886;-0.00012 -6.85779815965879e-07 428.663501196071 -684.578781865149;-0.0001 -6.91331316900679e-07 432.956346784322 -681.87191438129;-8e-05 -6.96855525258837e-07 437.232099997342 -679.138127761803;-6e-05 -7.02352222954065e-07 441.490592035716 -676.377529931902;-4e-05 -7.0782119298615e-07 445.731654781469 -673.590229875264;-2e-05 -7.13262219449521e-07 449.955120804706 -670.776337629722]  x5=0.000371346567279139  V1=[7.818e-10 4.235e+05 4.235e+05;314.2 314.2 314.2;1.708 0.8658 -0.705]  V2=[9.391e-10 4.188e+05 4.188e+05;314.2 314.2 314.2;1.235 0.8998 -0.671]  I1=[4.724e-12 1961 1961;314.2 314.2 314.2;-0.8175 0.9762 -0.5946]  I2=[5.7e-12 807.8 807.8;314.2 314.2 314.2;1.598 0.522 -1.049]  nHarmo=1  Measurements=None  Decoupling=off  VsMag0=0  VrMag0=0  VsAngle0=0  VrAngle0=0  IsMag0=0  IrMag0=0  IsAngle0=0  IrAngle0=0
      settings: SourceProductBaseCode=PS
  Line_69_b : spsDistributedParametersLineLib/Distributed Parameters Line  Phases=3  Length=70  Frequency=50  Resistance=[0.0298 0.1619]  Inductance=[1.0568e-03 3.9470e-03]  Capacitance=[11.0414e-09 7.1301e-09]  x1=[-0.00038 -0.000329257562447815 316167.901537245 -274630.335422951;-0.00036 -0.000330626020864734 317887.202585653 -272638.386013764;-0.00034 -0.000331981426732472 319593.953991614 -270635.673307929;-0.00032 -0.000333323726541925 321288.088375503 -268622.276369114;-0.0003 -0.000334652867301396 322969.538855796 -266598.274682783;-0.00028 -0.000335968796538684 324638.239051708 -264563.748153057;-0.00026 -0.000337271462303155 326294.123085812 -262518.77709956;-0.00024 -0.000338560813167795 327937.125586641 -260463.442254247;-0.00022 -0.000339836798231241 329567.181691271 -258397.824758218;-0.0002 -0.000341099367119786 331184.227047877 -256322.006158516;-0.00018 -0.000342348469989373 332788.197818277 -254236.068404905;-0.00016 -0.00034358405752756 334379.030680451 -252140.093846634;-0.00014 -0.000344806080955465 335956.662831044 -250034.165229192;-0.00012 -0.000346014492029696 337521.031987837 -247918.365691034;-0.0001 -0.000347209243044255 339072.076392217 -245792.778760302;-8e-05 -0.000348390286832415 340609.734811604 -243657.488351529;-6e-05 -0.00034955757676859 342133.946541879 -241512.578762325;-4e-05 -0.000350711066770174 343644.651409772 -239358.134670047;-2e-05 -0.000351850711299355 345141.78977524 -237194.241128459]  x2=[-0.00038 -0.00026869706755023 320559.87223326 -259085.932235473;-0.00036 -0.000270104539538551 322181.418864896 -257066.694275181;-0.00034 -0.000271501348262145 323790.246325777 -255037.307761968;-0.00032 -0.000272887438577394 325386.291102152 -252997.852812538;-0.0003 -0.000274262755763827 326969.490184904 -250948.40994108;-0.00028 -0.000275627245526274 328539.781072046 -248889.060056091;-0.00026 -0.000276980853997018 330097.101771181 -246819.884457176;-0.00024 -0.000278323527737913 331641.390801954 -244740.964831847;-0.00022 -0.0002796552137425 333172.58719848 -242652.38325229;-0.0002 -0.000280975859438094 334690.630511746 -240554.22217213;-0.00018 -0.000282285412687865 336195.460812002 -238446.564423173;-0.00016 -0.000283583821792893 337687.018691123 -236329.493212138;-0.00014 -0.000284871035494211 339165.24526496 -234203.092117373;-0.00012 -0.000286147002974824 340630.082175657 -232067.44508555;-0.0001 -0.000287411673861722 342081.471593962 -229922.636428359;-8e-05 -0.000288664998227864 343519.356221506 -227768.750819172;-6e-05 -0.000289906926594149 344943.679293066 -225605.873289705;-4e-05 -0.000291137409931372 346354.384578805 -223434.08922666;-2e-05 -0.000292356399662159 347751.416386495 -221253.484368353]  x3=[-0.00038 -2.63798158069164e-07 1662.23168875971 -1049.1674276373;-0.00036 -2.61548995041732e-07 1668.79094770687 -1038.70267696712;-0.00034 -2.5928950650782e-07 1675.28432564485 -1028.1969200938;-0.00032 -2.57019781668166e-07 1681.71156622619 -1017.65057176663;-0.0003 -2.54739910127619e-07 1688.07241571445 -1007.06404833738;-0.00028 -2.52449981891606e-07 1694.36662299418 -996.437767743874;-0.00026 -2.50150087362571e-07 1700.59393958085 -985.772149493471;-0.00024 -2.47840317336413e-07 1706.75411963067 -975.06761464652;-0.00022 -2.45520762998896e-07 1712.84691995028 -964.324585799725;-0.0002 -2.43191515922056e-07 1718.87210000636 -953.543487069471;-0.00018 -2.40852668060577e-07 1724.8294219351 -942.724744075075;-0.00016 -2.38504311748169e-07 1730.71865055165 -931.868783921987;-0.00014 -2.36146539693918e-07 1736.53955335934 -920.976035184924;-0.00012 -2.33779444978628e-07 1742.2919005589 -910.046927890955;-0.0001 -2.31403121051144e-07 1747.9754650575 -899.081893502524;-8e-05 -2.29017661724667e-07 1753.59002247776 -888.081364900412;-6e-05 -2.26623161173046e-07 1759.13535116656 -877.045776366652;-4e-05 -2.24219713927063e-07 1764.61123220381 -865.975563567385;-2e-05 -2.218074148707e-07 1770.01744941112 -854.871163535655]  x4=[-0.00038 -4.96186854934105e-07 320.889986448358 -744.354894952165;-0.00036 -5.02417918201012e-07 325.560541318688 -742.324004048294;-0.00034 -5.08629146868787e-07 330.218243616296 -740.263807463807;-0.00032 -5.14820295728756e-07 334.86290946307 -738.174386531735;-0.0003 -5.20991120364963e-07 339.494355495556 -736.05582373884;-0.00028 -5.27141377163817e-07 344.112398872194 -733.908202722353;-0.00026 -5.33270823323712e-07 348.716857280539 -731.731608266675;-0.00024 -5.39379216864608e-07 353.307548944458 -729.526126300027;-0.00022 -5.45466316637587e-07 357.884292631305 -727.291843891062;-0.0002 -5.51531882334373e-07 362.446907659074 -725.028849245424;-0.00018 -5.57575674496819e-07 366.995213903537 -722.737231702265;-0.00016 -5.63597454526358e-07 371.529031805351 -720.417081730723;-0.00014 -5.69596984693425e-07 376.04818237715 -718.068490926346;-0.00012 -5.75574028146843e-07 380.552487210606 -715.691552007478;-0.0001 -5.81528348923171e-07 385.041768483477 -713.286358811596;-8e-05 -5.87459711956019e-07 389.515848966626 -710.853006291611;-6e-05 -5.93367883085331e-07 393.974552031015 -708.391590512112;-4e-05 -5.99252629066628e-07 398.417701654683 -705.902208645581;-2e-05 -6.05113717580213e-07 402.845122429689 -703.38495896855]  x5=0.000371346567279139  V1=[9.514e-10 4.188e+05 4.188e+05;314.2 314.2 314.2;1.248 0.8998 -0.671]  V2=[3.385e-10 4.122e+05 4.122e+05;314.2 314.2 314.2;1.899 0.9353 -0.6355]  I1=[9.51e-12 1966 1966;314.2 314.2 314.2;2.181 1.052 -0.5188]  I2=[1.088e-11 810.7 810.7;314.2 314.2 314.2;-0.4113 0.4513 -1.119]  nHarmo=1  Measurements=None  Decoupling=off  VsMag0=0  VrMag0=0  VsAngle0=0  VrAngle0=0  IsMag0=0  IrMag0=0  IsAngle0=0  IrAngle0=0
      settings: SourceProductBaseCode=PS
  Line_78_a : spsDistributedParametersLineLib/Distributed Parameters Line  Phases=3  Length=100  Frequency=50  Resistance=[0.0298 0.1619]  Inductance=[1.0568e-03 3.9470e-03]  Capacitance=[11.0414e-09 7.1301e-09]  x1=[-0.00054 -7.85429295223008e-05 302306.562120962 -277089.977884906;-0.00052 -8.27243598145392e-05 304041.59106689 -275185.072715649;-0.0005 -8.69025242906988e-05 305764.616971406 -273269.303710913;-0.00048 -9.10772580040004e-05 307475.571812396 -271342.746501979;-0.00046 -9.52483961431053e-05 309174.388044294 -269405.477146025;-0.00044 -9.94157740386217e-05 310860.998600743 -267457.572123131;-0.00042 -0.000103579227169606 312535.336897247 -265499.108333249;-0.0004 -0.000107738591170058 314197.336833796 -263530.163093178;-0.00038 -0.000111893701835409 315846.932797479 -261550.814133504;-0.00036 -0.000116044395129004 317484.059665072 -259561.139595534;-0.00034 -0.000120190507188578 319108.652805609 -257561.218028213;-0.00032 -0.000124331874332729 320720.648082935 -255551.12838502;-0.0003 -0.00012846833306737 322319.981858236 -253530.950020852;-0.00028 -0.000132599720092196 323906.590992554 -251500.762688891;-0.00026 -0.000136725872307119 325480.412849276 -249460.646537458;-0.00024 -0.000140846626818716 327041.385296611 -247410.682106845;-0.00022 -0.000144961820946654 328589.446710038 -245350.950326136;-0.0002 -0.000149071292230115 330124.535974745 -243281.532510018;-0.00018 -0.00015317487843421 331646.592488035 -241202.51035556;-0.00016 -0.000157272417556382 333155.556161724 -239113.965938998;-0.00014 -0.000161363747832802 334651.367424509 -237015.98171249;-0.00012 -0.000165448707744757 336133.967224323 -234908.64050086;-0.0001 -0.000169527136025024 337603.297030665 -232792.025498331;-8e-05 -0.000173598871664237 339059.298836909 -230666.22026524;-6e-05 -0.000177663753917246 340501.915162598 -228531.308724736;-4e-05 -0.000181721622309459 341931.089055709 -226387.375159472;-2e-05 -0.000185772316643181 343346.764094904 -224234.504208274]  x2=[-0.00054 1.48739815183893e-05 278378.680791826 -309253.465693095;-0.00052 1.18417521602133e-05 280316.269878651 -307498.267967611;-0.0005 8.80905530993837e-06 282242.792559119 -305730.930737029;-0.00048 5.7760106932433e-06 284158.172777414 -303951.523772797;-0.00046 2.74273804953618e-06 286062.334917605 -302160.117322855;-0.00044 -2.90642872772819e-07 287955.20380663 -300356.782108862;-0.00042 -3.32401232099887e-06 289836.704717267 -298541.589323404;-0.0004 -6.35725054291011e-06 291706.763371082 -296714.610627185;-0.00038 -9.39023779145526e-06 293565.30594136 -294875.918146196;-0.00036 -1.24228543294911e-05 295412.259056025 -293025.584468866;-0.00034 -1.54549804345093e-05 297247.549800529 -291163.682643201;-0.00032 -1.84864964033631e-05 299071.105720736 -289290.286173898;-0.0003 -2.15172825569929e-05 300882.854825781 -287405.469019441;-0.00028 -2.45472192451508e-05 302682.725590912 -285509.305589185;-0.00026 -2.75761868511245e-05 304470.646960312 -283601.870740413;-0.00024 -3.06040657964593e-05 306246.548349907 -281683.23977539;-0.00022 -3.3630736545679e-05 308010.359650151 -279753.488438378;-0.0002 -3.66560796110049e-05 309762.011228795 -277812.692912658;-0.00018 -3.9679975557073e-05 311501.433933633 -275860.929817514;-0.00016 -4.27023050056492e-05 313228.559095235 -273898.276205209;-0.00014 -4.57229486403418e-05 314943.318529657 -271924.809557949;-0.00012 -4.87417872113123e-05 316645.644541133 -269940.607784818;-0.0001 -5.1758701539983e-05 318335.469924747 -267945.749218703;-8e-05 -5.4773572523742e-05 320012.727969086 -265940.312613206;-6e-05 -5.77862811406451e-05 321677.352458874 -263924.37713953;-4e-05 -6.07967084541148e-05 323329.277677586 -261898.022383355;-2e-05 -6.38047356176353e-05 324968.438410045 -259861.328341698]  x3=[-0.00054 -1.37811434507393e-06 -99.8580702469036 -314.330210210326;-0.00052 -1.37786978526755e-06 -97.8811171717715 -314.95142821796;-0.0005 -1.37757082952134e-06 -95.9002999177329 -315.560212482492;-0.00048 -1.37721748963755e-06 -93.9156966840611 -316.15653897016;-0.00046 -1.37680977956545e-06 -91.9273858194937 -316.740384139016;-0.00044 -1.37634771540073e-06 -89.935445819139 -317.311724939853;-0.00042 -1.37583131538489e-06 -87.9399553213776 -317.870538817114;-0.0004 -1.37526059990452e-06 -85.9409931047573 -318.416803709785;-0.00038 -1.37463559149048e-06 -83.9386380848838 -318.950498052261;-0.00036 -1.37395631481705e-06 -81.9329693113047 -319.471600775205;-0.00034 -1.3732227967009e-06 -79.924065964389 -319.980091306374;-0.00032 -1.37243506610007e-06 -77.9120073522008 -320.475949571431;-0.0003 -1.37159315411281e-06 -75.8968729073691 -320.959155994742;-0.00028 -1.37069709397638e-06 -73.8787421839514 -321.429691500145;-0.00026 -1.36974692106568e-06 -71.8576948542928 -321.887537511703;-0.00024 -1.36874267289192e-06 -69.8338107058815 -322.332675954439;-0.00022 -1.3676843891011e-06 -67.8071696381981 -322.765089255051;-0.0002 -1.36657211147245e-06 -65.7778516595619 -323.184760342602;-0.00018 -1.36540588391678e-06 -63.7459368839719 -323.591672649195;-0.00016 -1.36418575247477e-06 -61.7115055279443 -323.985810110629;-0.00014 -1.36291176531511e-06 -59.6746379073454 -324.367157167033;-0.00012 -1.36158397273263e-06 -57.6354144342213 -324.735698763478;-0.0001 -1.36020242714631e-06 -55.593915613623 -325.091420350572;-8e-05 -1.35876718309721e-06 -53.5502220404283 -325.434307885036;-6e-05 -1.35727829724631e-06 -51.5044143961601 -325.764347830258;-4e-05 -1.35573582837226e-06 -49.4565734458012 -326.081527156825;-2e-05 -1.3541398373691e-06 -47.4067800346059 -326.385833343041]  x4=[-0.00054 1.42144140306474e-06 1862.00305986408 -1667.60028866092;-0.00052 1.41161158085589e-06 1872.44407818777 -1655.86813839409;-0.0005 1.4017260306389e-06 1882.81117562539 -1644.07061728846;-0.00048 1.39178514267836e-06 1893.10394290168 -1632.20819108995;-0.00046 1.3817893094235e-06 1903.32197367582 -1620.28132810685;-0.00044 1.37173892549271e-06 1913.46486455746 -1608.29049919128;-0.00042 1.36163438765794e-06 1923.53221512261 -1596.23617772064;-0.0004 1.35147609482903e-06 1933.52362792953 -1584.11883957889;-0.00038 1.34126444803799e-06 1943.43870853434 -1571.93896313781;-0.00036 1.33099985042316e-06 1953.27706550663 -1559.69702923804;-0.00034 1.32068270721327e-06 1963.03831044493 -1547.3935211702;-0.00032 1.31031342571147e-06 1972.72205799199 -1535.0289246557;-0.0003 1.29989241527924e-06 1982.32792585004 -1522.60372782765;-0.00028 1.28942008732023e-06 1991.85553479586 -1510.11842121153;-0.00026 1.27889685526401e-06 2001.30450869578 -1497.57349770589;-0.00024 1.26832313454977e-06 2010.67447452048 -1484.96945256281;-0.00022 1.25769934260989e-06 2019.96506235974 -1472.30678336842;-0.0002 1.24702589885349e-06 2029.17590543708 -1459.58599002321;-0.00018 1.23630322464986e-06 2038.30664012418 -1446.80757472233;-0.00016 1.2255317433118e-06 2047.35690595527 -1433.97204193573;-0.00014 1.21471188007897e-06 2056.32634564135 -1421.07989838827;-0.00012 1.20384406210103e-06 2065.21460508429 -1408.1316530397;-0.0001 1.19292871842083e-06 2074.02133339084 -1395.12781706458;-8e-05 1.18196627995745e-06 2082.74618288644 -1382.06890383208;-6e-05 1.17095717948919e-06 2091.38880912898 -1368.95542888573;-4e-05 1.15990185163648e-06 2099.94887092236 -1355.78790992308;-2e-05 1.14880073284473e-06 2108.42603033 -1342.56686677523]  x5=0.000530495096113056  V1=[8.92e-10 4.101e+05 4.101e+05;314.2 314.2 314.2;-0.7547 0.8912 -0.6796]  V2=[4.527e-10 4.161e+05 4.161e+05;314.2 314.2 314.2;-0.9521 0.7952 -0.7756]  I1=[5.472e-12 329.9 329.9;314.2 314.2 314.2;0.6215 -0.2451 -1.816]  I2=[4.185e-12 2499 2499;314.2 314.2 314.2;-1.63 0.9027 -0.6681]  nHarmo=1  Measurements=None  Decoupling=off  VsMag0=0  VrMag0=0  VsAngle0=0  VrAngle0=0  IsMag0=0  IrMag0=0  IsAngle0=0  IrAngle0=0
      settings: SourceProductBaseCode=PS
  Line_78_b : spsDistributedParametersLineLib/Distributed Parameters Line  Phases=3  Length=10  Frequency=50  Resistance=[0.0298 0.1619]  Inductance=[1.0568e-03 3.9470e-03]  Capacitance=[11.0414e-09 7.1301e-09]  x1=[-6e-05 -5.77862668655959e-05 0 0;-4e-05 -6.07966940862085e-05 323329.277677586 -261898.022383355;-2e-05 -6.38047211574391e-05 324968.438410045 -259861.328341698]  x2=[-6e-05 -4.57637226826741e-05 0 0;-4e-05 -4.86641854669159e-05 321274.746392595 -265271.00478101;-2e-05 -5.15627270724418e-05 322935.140613804 -263247.153075453]  x3=[-6e-05 -1.33716223973438e-06 0 0;-4e-05 -1.33405770046815e-06 -22.6246355825345 -328.352569324679;-2e-05 -1.33090049488817e-06 -20.5611025242458 -328.488241753983]  x4=[-6e-05 1.20873908960229e-06 0 0;-4e-05 1.19769546757575e-06 2095.55401595842 -1385.57568109593;-2e-05 1.18660456258293e-06 2104.21842297154 -1372.38166346976]  x5=5.30495096113055e-05  V1=[4.527e-10 4.161e+05 4.161e+05;314.2 314.2 314.2;-0.8021 0.8918 -0.679]  V2=[3.459e-10 4.166e+05 4.166e+05;314.2 314.2 314.2;-1.332 0.8824 -0.6884]  I1=[2.305e-11 329.2 329.2;314.2 314.2 314.2;1.554 -0.06674 -1.638]  I2=[1.894e-11 2512 2512;314.2 314.2 314.2;-2.04 0.9884 -0.5824]  nHarmo=1  Measurements=None  Decoupling=off  VsMag0=0  VrMag0=0  VsAngle0=0  VrAngle0=0  IsMag0=0  IrMag0=0  IsAngle0=0  IrAngle0=0
      settings: SourceProductBaseCode=PS
  Line_89_a : spsDistributedParametersLineLib/Distributed Parameters Line  Phases=3  Length=100  Frequency=50  Resistance=[0.0298 0.1619]  Inductance=[1.0568e-03 3.9470e-03]  Capacitance=[11.0414e-09 7.1301e-09]  x1=[-0.00054 2.4092731032811e-05 275822.518800151 -312264.781068341;-0.00052 2.11805631268812e-05 277779.078871523 -310525.584635892;-0.0005 1.8267559048586e-05 279724.672700495 -308774.129185066;-0.00048 1.53538337983387e-05 281659.223478353 -307010.483860326;-0.00046 1.2439502405023e-05 283582.654832347 -305234.71828737;-0.00044 9.52467992145222e-06 285494.890828699 -303446.902570381;-0.00042 6.60948141982697e-06 287395.855975607 -301647.107289263;-0.0004 3.69402198719251e-06 289285.475226221 -299835.403496852;-0.00038 7.78416720895187e-07 291163.67398161 -298011.862716111;-0.00036 -2.13721927596143e-06 293030.378093702 -296176.556937308;-0.00034 -5.05277089906052e-06 294885.513868215 -294329.558615173;-0.00032 -7.96812304741626e-06 296729.008067565 -292470.940666036;-0.0003 -1.08831606279177e-05 298560.787913758 -290600.776464953;-0.00028 -1.37977685598725e-05 300380.781091263 -288719.139842803;-0.00026 -1.67118317795501e-05 302188.915749864 -286826.105083378;-0.00024 -1.96252352447243e-05 303985.120507502 -284921.74692045;-0.00022 -2.25378639392148e-05 305769.324453088 -283006.140534817;-0.0002 -2.54496028774281e-05 307541.457149305 -281079.36155134;-0.00018 -2.83603371088964e-05 309301.44863539 -279141.486035954;-0.00016 -3.12699517228163e-05 311049.229429891 -277192.590492666;-0.00014 -3.41783318525849e-05 312784.730533416 -275232.751860535;-0.00012 -3.70853626803347e-05 314507.883431353 -273262.047510635;-0.0001 -3.99909294414662e-05 316218.620096576 -271280.555242998;-8e-05 -4.28949174291787e-05 317916.87299213 -269288.353283548;-6e-05 -4.57972119989991e-05 319602.5750739 -267285.520281005;-4e-05 -4.8697698573307e-05 321275.659793253 -265272.135303787;-2e-05 -5.15962626458592e-05 322936.061099669 -263248.277836887]  x2=[-0.00054 -0.000231512612293426 304442.004312454 -278441.271086263;-0.00052 -0.000233130945140434 306185.481477516 -276522.921952887;-0.0005 -0.000234740074376912 307916.870964043 -274593.656168035;-0.00048 -0.000236339936477192 309636.104419742 -272653.549895817;-0.00046 -0.00023793046828146 311343.11397222 -270702.679728307;-0.00044 -0.000239511606998242 313037.832231664 -268741.122682518;-0.00042 -0.000241083290206889 314720.192293498 -266768.956197365;-0.0004 -0.00024264545586004 316390.127741027 -264786.258130602;-0.00038 -0.000244198042286069 318047.57264806 -262793.106755756;-0.00036 -0.000245740988191522 319692.461581509 -260789.580759028;-0.00034 -0.000247274232663537 321324.729603976 -258775.759236195;-0.00032 -0.000248797715172249 322944.312276315 -256751.721689483;-0.0003 -0.000250311375573175 324551.145660174 -254717.548024427;-0.00028 -0.000251815154109595 326145.166320523 -252673.318546722;-0.00026 -0.000253308991414908 327726.311328155 -250619.113959047;-0.00024 -0.000254792828514974 329294.518262174 -248555.015357882;-0.00022 -0.000256266606830446 330849.725212454 -246481.104230304;-0.0002 -0.000257730268179078 332391.870782089 -244397.462450775;-0.00018 -0.000259183754778028 333920.894089811 -242304.172277903;-0.00016 -0.000260627009246133 335436.734772398 -240201.316351201;-0.00014 -0.000262059974606177 336939.332987056 -238088.977687821;-0.00012 -0.000263482594287143 338428.629413781 -235967.239679274;-0.0001 -0.000264894812126441 339904.565257699 -233836.186088146;-8e-05 -0.000266296572372128 341367.08225139 -231695.901044783;-6e-05 -0.000267687819685112 342816.122657188 -229546.469043973;-4e-05 -0.000269068499141329 344251.629269459 -227387.974941612;-2e-05 -0.000270438556233918 345673.54541686 -225220.503951351]  x3=[-0.00054 -1.79466580969218e-06 1915.25413349812 -1812.17366647108;-0.00052 -1.80980201190479e-06 1926.60247603913 -1800.10407825351;-0.0005 -1.82486676623284e-06 1937.87475961325 -1787.96342500921;-0.00048 -1.83985947794564e-06 1949.07053921004 -1775.75218603037;-0.00046 -1.85477955515659e-06 1960.18937283928 -1763.4708433958;-0.00044 -1.86962640884659e-06 1971.23082154846 -1751.11988195188;-0.00042 -1.88439945288729e-06 1982.1944494401 -1738.69978929342;-0.0004 -1.89909810406419e-06 1993.07982368893 -1726.2110557444;-0.00038 -1.91372178209972e-06 2003.88651455902 -1713.65417433865;-0.00036 -1.92826990967611e-06 2014.61409542072 -1701.02964080035;-0.00034 -1.9427419124582e-06 2025.26214276751 -1688.33795352446;-0.00032 -1.95713721911609e-06 2035.8302362327 -1675.57961355705;-0.0003 -1.97145526134772e-06 2046.31795860607 -1662.75512457556;-0.00028 -1.98569547390131e-06 2056.72489585029 -1649.86499286884;-0.00026 -1.99985729459764e-06 2067.0506371173 -1636.90972731723;-0.00024 -2.01394016435229e-06 2077.29477476451 -1623.88983937241;-0.00022 -2.02794352719766e-06 2087.45690437091 -1610.80584303729;-0.0002 -2.04186683030498e-06 2097.53662475303 -1597.65825484562;-0.00018 -2.05570952400607e-06 2107.53353798076 -1584.44759384168;-0.00016 -2.06947106181509e-06 2117.44724939309 -1571.17438155975;-0.00014 -2.0831509004501e-06 2127.27736761366 -1557.83914200351;-0.00012 -2.09674849985448e-06 2137.02350456623 -1544.44240162539;-0.0001 -2.11026332321829e-06 2146.68527549002 -1530.98468930577;-8e-05 -2.12369483699946e-06 2156.26229895485 -1517.46653633208;-6e-05 -2.13704251094481e-06 2165.75419687623 -1503.88847637785;-4e-05 -2.15030581811102e-06 2175.16059453028 -1490.25104548164;-2e-05 -2.16348423488546e-06 2184.48112056852 -1476.55478202588]  x4=[-0.00054 1.60054680610595e-06 -155.212984478826 -183.683972205365;-0.00052 1.60954622276162e-06 -154.055807864468 -184.655571987055;-0.0005 1.6184820972884e-06 -152.8925493906 -185.619881882945;-0.00048 1.62735407691326e-06 -151.723254980677 -186.57686382373;-0.00046 1.63616181138565e-06 -150.547970796439 -187.526480029402;-0.00044 1.64490495299127e-06 -149.366743236093 -188.468693010739;-0.00042 1.65358315656589e-06 -148.179618932482 -189.403465570787;-0.0004 1.66219607950886e-06 -146.986644751238 -190.330760806324;-0.00038 1.67074338179676e-06 -145.787867788942 -191.250542109323;-0.00036 1.67922472599671e-06 -144.583335371254 -192.162773168393;-0.00034 1.68763977727978e-06 -143.373095051052 -193.067417970214;-0.00032 1.69598820343414e-06 -142.157194606551 -193.964440800957;-0.0003 1.70426967487822e-06 -140.93568203942 -194.853806247698;-0.00028 1.71248386467372e-06 -139.708605572882 -195.735479199812;-0.00026 1.72063044853848e-06 -138.476013649815 -196.609424850359;-0.00024 1.72870910485932e-06 -137.237954930838 -197.475608697463;-0.00022 1.73671951470473e-06 -135.99447829239 -198.333996545668;-0.0002 1.74466136183744e-06 -134.745632824799 -199.184554507291;-0.00018 1.75253433272692e-06 -133.491467830345 -200.027249003761;-0.00016 1.76033811656177e-06 -132.232032821315 -200.862046766942;-0.00014 1.76807240526195e-06 -130.967377518047 -201.688914840447;-0.00012 1.775736893491e-06 -129.697551846967 -202.507820580941;-0.0001 1.78333127866805e-06 -128.422605938617 -203.318731659428;-8e-05 1.79085526097976e-06 -127.14259012568 -204.121616062526;-6e-05 1.79830854339221e-06 -125.857554940988 -204.916442093734;-4e-05 1.80569083166256e-06 -124.567551115529 -205.703178374682;-2e-05 1.81300183435071e-06 -123.272629576446 -206.481793846367]  x5=0.000530495096113056  V1=[5.499e-10 4.166e+05 4.166e+05;314.2 314.2 314.2;-1.286 0.7858 -0.785]  V2=[5.945e-10 4.126e+05 4.126e+05;314.2 314.2 314.2;-0.5426 0.8923 -0.6785]  I1=[4.251e-12 2637 2637;314.2 314.2 314.2;-0.8207 0.8753 -0.6955]  I2=[3.147e-12 240.5 240.5;314.2 314.2 314.2;2.253 -0.6397 -2.211]  nHarmo=1  Measurements=None  Decoupling=off  VsMag0=0  VrMag0=0  VsAngle0=0  VrAngle0=0  IsMag0=0  IrMag0=0  IsAngle0=0  IrAngle0=0
      settings: SourceProductBaseCode=PS
  Line_89_b : spsDistributedParametersLineLib/Distributed Parameters Line  Phases=3  Length=10  Frequency=50  Resistance=[0.0298 0.1619]  Inductance=[1.0568e-03 3.9470e-03]  Capacitance=[11.0414e-09 7.1301e-09]  x1=[-6e-05 -0.000267687819753682 0 0;-4e-05 -0.000269068499187044 344251.629269459 -227387.974941612;-2e-05 -0.000270438556256776 345673.54541686 -225220.503951351]  x2=[-6e-05 -0.000289631923134944 0 0;-4e-05 -0.000290857574281786 346349.132928433 -223429.070806512;-2e-05 -0.000292071742869623 347746.133308335 -221248.499044142]  x3=[-6e-05 -2.53266982458721e-06 0 0;-4e-05 -2.54382116703603e-06 2346.56712034886 -1260.7396304865;-2e-05 -2.55487208378089e-06 2354.44220970815 -1245.97092550921]  x4=[-6e-05 1.78947207468638e-06 0 0;-4e-05 1.79708679751395e-06 -123.74486939869 -207.369435651975;-2e-05 1.80463057443186e-06 -122.439494764109 -208.142849205593]  x5=5.30495096113055e-05  V1=[5.916e-10 4.126e+05 4.126e+05;314.2 314.2 314.2;-0.4212 0.9888 -0.582]  V2=[6.139e-10 4.122e+05 4.122e+05;314.2 314.2 314.2;-0.1116 0.9997 -0.5711]  I1=[1.499e-11 2664 2664;314.2 314.2 314.2;1.83 1.08 -0.4912]  I2=[2.162e-11 241.5 241.5;314.2 314.2 314.2;2.618 -0.5367 -2.107]  nHarmo=1  Measurements=None  Decoupling=off  VsMag0=0  VrMag0=0  VsAngle0=0  VrAngle0=0  IsMag0=0  IrMag0=0  IsAngle0=0  IrAngle0=0
      settings: SourceProductBaseCode=PS
  Ln_45 : spsThreePhaseVIMeasurementLib/Three-Phase V-I Measurement  VoltageMeasurement=phase-to-ground  SetLabelV=on  LabelV=Vabc_Ln_45  Vpu=off  VpuLL=off  CurrentMeasurement=yes  SetLabelI=on  LabelI=Iabc_Ln_45  Ipu=off  Pbase=100e6  Vbase=500e3  OutputType=Complex  PhasorSimulation=off  PSBequivalent=0
  Ln_46 : spsThreePhaseVIMeasurementLib/Three-Phase V-I Measurement  VoltageMeasurement=phase-to-ground  SetLabelV=on  LabelV=Vabc_Ln_46  Vpu=off  VpuLL=off  CurrentMeasurement=yes  SetLabelI=on  LabelI=Iabc_Ln_46  Ipu=off  Pbase=100e6  Vbase=500e3  OutputType=Complex  PhasorSimulation=off  PSBequivalent=0
  Ln_54 : spsThreePhaseVIMeasurementLib/Three-Phase V-I Measurement  VoltageMeasurement=phase-to-ground  SetLabelV=on  LabelV=Vabc_Ln_54  Vpu=off  VpuLL=off  CurrentMeasurement=yes  SetLabelI=on  LabelI=Iabc_Ln_54  Ipu=off  Pbase=100e6  Vbase=500e3  OutputType=Complex  PhasorSimulation=off  PSBequivalent=0
  Ln_57 : spsThreePhaseVIMeasurementLib/Three-Phase V-I Measurement  VoltageMeasurement=phase-to-ground  SetLabelV=on  LabelV=Vabc_Ln_57  Vpu=off  VpuLL=off  CurrentMeasurement=yes  SetLabelI=on  LabelI=Iabc_Ln_57  Ipu=off  Pbase=100e6  Vbase=500e3  OutputType=Complex  PhasorSimulation=off  PSBequivalent=0
  Ln_64 : spsThreePhaseVIMeasurementLib/Three-Phase V-I Measurement  VoltageMeasurement=phase-to-ground  SetLabelV=on  LabelV=Vabc_Ln_64  Vpu=off  VpuLL=off  CurrentMeasurement=yes  SetLabelI=on  LabelI=Iabc_Ln_64  Ipu=off  Pbase=100e6  Vbase=500e3  OutputType=Complex  PhasorSimulation=off  PSBequivalent=0
  Ln_69 : spsThreePhaseVIMeasurementLib/Three-Phase V-I Measurement  VoltageMeasurement=phase-to-ground  SetLabelV=on  LabelV=Vabc_Ln_69  Vpu=off  VpuLL=off  CurrentMeasurement=yes  SetLabelI=on  LabelI=Iabc_Ln_69  Ipu=off  Pbase=100e6  Vbase=500e3  OutputType=Complex  PhasorSimulation=off  PSBequivalent=0
  Ln_75 : spsThreePhaseVIMeasurementLib/Three-Phase V-I Measurement  VoltageMeasurement=phase-to-ground  SetLabelV=on  LabelV=Vabc_Ln_75  Vpu=off  VpuLL=off  CurrentMeasurement=yes  SetLabelI=on  LabelI=Iabc_Ln_75  Ipu=off  Pbase=100e6  Vbase=500e3  OutputType=Complex  PhasorSimulation=off  PSBequivalent=0
  Ln_78 : spsThreePhaseVIMeasurementLib/Three-Phase V-I Measurement  VoltageMeasurement=phase-to-ground  SetLabelV=on  LabelV=Vabc_Ln_78  Vpu=off  VpuLL=off  CurrentMeasurement=yes  SetLabelI=on  LabelI=Iabc_Ln_78  Ipu=off  Pbase=100e6  Vbase=500e3  OutputType=Complex  PhasorSimulation=off  PSBequivalent=0
  Ln_87 : spsThreePhaseVIMeasurementLib/Three-Phase V-I Measurement  VoltageMeasurement=phase-to-ground  SetLabelV=on  LabelV=Vabc_Ln_87  Vpu=off  VpuLL=off  CurrentMeasurement=yes  SetLabelI=on  LabelI=Iabc_Ln_87  Ipu=off  Pbase=100e6  Vbase=500e3  OutputType=Complex  PhasorSimulation=off  PSBequivalent=0
  Ln_89 : spsThreePhaseVIMeasurementLib/Three-Phase V-I Measurement  VoltageMeasurement=phase-to-ground  SetLabelV=on  LabelV=Vabc_Ln_89  Vpu=off  VpuLL=off  CurrentMeasurement=yes  SetLabelI=on  LabelI=Iabc_Ln_89  Ipu=off  Pbase=100e6  Vbase=500e3  OutputType=Complex  PhasorSimulation=off  PSBequivalent=0
  Ln_96 : spsThreePhaseVIMeasurementLib/Three-Phase V-I Measurement  VoltageMeasurement=phase-to-ground  SetLabelV=on  LabelV=Vabc_Ln_96  Vpu=off  VpuLL=off  CurrentMeasurement=yes  SetLabelI=on  LabelI=Iabc_Ln_96  Ipu=off  Pbase=100e6  Vbase=500e3  OutputType=Complex  PhasorSimulation=off  PSBequivalent=0
  Ln_98 : spsThreePhaseVIMeasurementLib/Three-Phase V-I Measurement  VoltageMeasurement=phase-to-ground  SetLabelV=on  LabelV=Vabc_Ln_98  Vpu=off  VpuLL=off  CurrentMeasurement=yes  SetLabelI=on  LabelI=Iabc_Ln_98  Ipu=off  Pbase=100e6  Vbase=500e3  OutputType=Complex  PhasorSimulation=off  PSBequivalent=0
  "Load A 1020 MW, 320 MVAR" : spsThreePhaseParallelRLCLoadLib/Three-Phase Parallel RLC Load  LConnTagsString=A|B|C  Configuration=Y (grounded)  NominalVoltage=(400000)*1.04156  Vabc=[1e3 1e3 1e3]  Vabcp=[1e3 1e3 1e3]  NominalFrequency=50  UnbalancedPower=off  ActivePower=1020000000  InductivePower=320000000  CapacitivePower=0  Pabc=[10e3 9e3 11e3]  QLabc=[100 90 110]  QCabc=[100 90 110]  Pabcp=[10e3 9e3 11e3]  QLabcp=[100 90 110]  QCabcp=[100 90 110]  Measurements=None  LoadType=constant PQ
  "Load B 850 MW, 250 MVAR" : spsThreePhaseParallelRLCLoadLib/Three-Phase Parallel RLC Load  LConnTagsString=A|B|C  Configuration=Y (grounded)  NominalVoltage=(400000)*1.05047  Vabc=[1e3 1e3 1e3]  Vabcp=[1e3 1e3 1e3]  NominalFrequency=50  UnbalancedPower=off  ActivePower=850000000  InductivePower=280000000  CapacitivePower=0  Pabc=[10e3 9e3 11e3]  QLabc=[100 90 110]  QCabc=[100 90 110]  Pabcp=[10e3 9e3 11e3]  QLabcp=[100 90 110]  QCabcp=[100 90 110]  Measurements=None  LoadType=constant PQ
  "Load C 360 MW, 120 MVAR" : spsThreePhaseParallelRLCLoadLib/Three-Phase Parallel RLC Load  LConnTagsString=A|B|C  Configuration=Y (grounded)  NominalVoltage=(400000)*1.05886  Vabc=[1e3 1e3 1e3]  Vabcp=[1e3 1e3 1e3]  NominalFrequency=50  UnbalancedPower=off  ActivePower=360000000  InductivePower=120000000  CapacitivePower=0  Pabc=[10e3 9e3 11e3]  QLabc=[100 90 110]  QCabc=[100 90 110]  Pabcp=[10e3 9e3 11e3]  QLabcp=[100 90 110]  QCabcp=[100 90 110]  Measurements=None  LoadType=constant PQ
  Load Flow Bus : spsLoadFlowBusLib/Load Flow Bus  LConnTagsString=a  Phases=single  Connectors=on one side  ID=BUS_1  Vbase=24e3  Vref=1  Vangle=0  VLF=1  VLFb=1  VLFc=1  angleLF=0  angleLFb=0  angleLFc=0
      settings: SourceProductBaseCode=PS
  Load Flow Bus1 : spsLoadFlowBusLib/Load Flow Bus  LConnTagsString=a  Phases=single  Connectors=on one side  ID=BUS_4  Vbase=400e3  Vref=1  Vangle=0  VLF=1.038  VLFb=1  VLFc=1  angleLF=25.46  angleLFb=0  angleLFc=0
      settings: SourceProductBaseCode=PS
  Load Flow Bus2 : spsLoadFlowBusLib/Load Flow Bus  LConnTagsString=a  Phases=single  Connectors=on one side  ID=BUS_5  Vbase=400e3  Vref=1  Vangle=0  VLF=1.05  VLFb=1  VLFc=1  angleLF=20.03  angleLFb=0  angleLFc=0
      settings: SourceProductBaseCode=PS
  Load Flow Bus3 : spsLoadFlowBusLib/Load Flow Bus  LConnTagsString=a  Phases=single  Connectors=on one side  ID=BUS_2  Vbase=26e3  Vref=1  Vangle=0  VLF=1  VLFb=1  VLFc=1  angleLF=4.046  angleLFb=0  angleLFc=0
      settings: SourceProductBaseCode=PS
  Load Flow Bus4 : spsLoadFlowBusLib/Load Flow Bus  LConnTagsString=a  Phases=single  Connectors=on one side  ID=BUS_7  Vbase=400e3  Vref=1  Vangle=0  VLF=1.025  VLFb=1  VLFc=1  angleLF=27.21  angleLFb=0  angleLFc=0
      settings: SourceProductBaseCode=PS
  Load Flow Bus5 : spsLoadFlowBusLib/Load Flow Bus  LConnTagsString=a  Phases=single  Connectors=on one side  ID=BUS_8  Vbase=400e3  Vref=1  Vangle=0  VLF=1.042  VLFb=1  VLFc=1  angleLF=21.17  angleLFb=0  angleLFc=0
      settings: SourceProductBaseCode=PS
  Load Flow Bus6 : spsLoadFlowBusLib/Load Flow Bus  LConnTagsString=a  Phases=single  Connectors=on one side  ID=BUS_9  Vbase=400e3  Vref=1  Vangle=0  VLF=1.03  VLFb=1  VLFc=1  angleLF=27.89  angleLFb=0  angleLFc=0
      settings: SourceProductBaseCode=PS
  Load Flow Bus7 : spsLoadFlowBusLib/Load Flow Bus  LConnTagsString=a  Phases=single  Connectors=on one side  ID=BUS_3  Vbase=26e3  Vref=1  Vangle=0  VLF=1  VLFb=1  VLFc=1  angleLF=4.557  angleLFb=0  angleLFc=0
      settings: SourceProductBaseCode=PS
  Load Flow Bus8 : spsLoadFlowBusLib/Load Flow Bus  LConnTagsString=a  Phases=single  Connectors=on one side  ID=BUS_6  Vbase=400e3  Vref=1  Vangle=0  VLF=1.059  VLFb=1  VLFc=1  angleLF=23.91  angleLFb=0  angleLFc=0
      settings: SourceProductBaseCode=PS
  Rotor Angle Deviations : Scope  Commented=on  NumInputPorts=2
  Scope : Scope  NumInputPorts=2
  Scope1 : Scope  Commented=on  NumInputPorts=3
  Scope2 : Scope  NumInputPorts=2
  Shunt Compensation 200 MVAr : spsThreePhaseParallelRLCLoadLib/Three-Phase Parallel RLC Load  LConnTagsString=A|B|C  Configuration=Y (grounded)  NominalVoltage=(400000)*0.905282  Vabc=[1e3 1e3 1e3]  Vabcp=[1e3 1e3 1e3]  NominalFrequency=50  UnbalancedPower=off  ActivePower=0  InductivePower=0  CapacitivePower=200000000  Pabc=[10e3 9e3 11e3]  QLabc=[100 90 110]  QCabc=[100 90 110]  Pabcp=[10e3 9e3 11e3]  QLabcp=[100 90 110]  QCabcp=[100 90 110]  Measurements=None  LoadType=constant Z
  Shunt Compensation 350 MVAr : spsThreePhaseParallelRLCLoadLib/Three-Phase Parallel RLC Load  LConnTagsString=A|B|C  Configuration=Y (grounded)  NominalVoltage=(400000)*0.905282  Vabc=[1e3 1e3 1e3]  Vabcp=[1e3 1e3 1e3]  NominalFrequency=50  UnbalancedPower=off  ActivePower=0  InductivePower=0  CapacitivePower=350000000  Pabc=[10e3 9e3 11e3]  QLabc=[100 90 110]  QCabc=[100 90 110]  Pabcp=[10e3 9e3 11e3]  QLabcp=[100 90 110]  QCabcp=[100 90 110]  Measurements=None  LoadType=constant Z
  Shunt Compensation 400 MVAr : spsThreePhaseParallelRLCLoadLib/Three-Phase Parallel RLC Load  LConnTagsString=A|B|C  Configuration=Y (grounded)  NominalVoltage=(400000)*0.905282  Vabc=[1e3 1e3 1e3]  Vabcp=[1e3 1e3 1e3]  NominalFrequency=50  UnbalancedPower=off  ActivePower=0  InductivePower=0  CapacitivePower=400000000  Pabc=[10e3 9e3 11e3]  QLabc=[100 90 110]  QCabc=[100 90 110]  Pabcp=[10e3 9e3 11e3]  QLabcp=[100 90 110]  QCabcp=[100 90 110]  Measurements=None  LoadType=constant Z
  Snb_G1 : spsThreePhaseSeriesRLCLoadLib/Three-Phase Series RLC Load  LConnTagsString=A|B|C  Configuration=Y (grounded)  NominalVoltage=26e3  Vabc=[1e3 1e3 1e3]  Vabcp=[1e3 1e3 1e3]  NominalFrequency=50  UnbalancedPower=off  ActivePower=1000000  InductivePower=0  CapacitivePower=10000000  Pabc=[10e3 9e3 11e3]  QLabc=[100 90 110]  QCabc=[100 90 110]  Pabcp=[10e3 9e3 11e3]  QLabcp=[100 90 110]  QCabcp=[100 90 110]  Measurements=None  LoadType=constant Z
  Snb_G2 : spsThreePhaseSeriesRLCLoadLib/Three-Phase Series RLC Load  LConnTagsString=A|B|C  Configuration=Y (grounded)  NominalVoltage=26e3  Vabc=[1e3 1e3 1e3]  Vabcp=[1e3 1e3 1e3]  NominalFrequency=50  UnbalancedPower=off  ActivePower=1000000  InductivePower=0  CapacitivePower=10000000  Pabc=[10e3 9e3 11e3]  QLabc=[100 90 110]  QCabc=[100 90 110]  Pabcp=[10e3 9e3 11e3]  QLabcp=[100 90 110]  QCabcp=[100 90 110]  Measurements=None  LoadType=constant Z
  Snb_G3 : spsThreePhaseSeriesRLCLoadLib/Three-Phase Series RLC Load  LConnTagsString=A|B|C  Configuration=Y (grounded)  NominalVoltage=26e3  Vabc=[1e3 1e3 1e3]  Vabcp=[1e3 1e3 1e3]  NominalFrequency=50  UnbalancedPower=off  ActivePower=1000000  InductivePower=0  CapacitivePower=10000000  Pabc=[10e3 9e3 11e3]  QLabc=[100 90 110]  QCabc=[100 90 110]  Pabcp=[10e3 9e3 11e3]  QLabcp=[100 90 110]  QCabcp=[100 90 110]  Measurements=None  LoadType=constant Z
  Source 1 776.5MVA,24kV,50Hz1 : spsThreePhaseSourceLib/Three-Phase Source  InternalConnection=Yg  VoltagePhases=off  Voltage=(24000)*1.02752  PhaseAngle=35.9818  Voltage_phases=[25e3 25e3 25e3]/sqrt(3)  PhaseAngles_phases=[0 -120 +120]  Frequency=50  NonIdealSource=on  SpecifyImpedance=on  Resistance=0.8929  Inductance=16.58e-3  ShortCircuitLevel=776.5e6  BaseVoltage=24e3  XRratio=7  BusType=swing  Pref=1020000000  Qref=0  Prefabc=[10e3, 10e3, 10e3]  Qrefabc=[0, 0, 0]  Qmin=-Inf  Qmax=Inf
  Source 2 1200MVA,26kV,50Hz : spsThreePhaseSourceLib/Three-Phase Source  InternalConnection=Yg  VoltagePhases=off  Voltage=(26000)*1.31746  PhaseAngle=45.2983  Voltage_phases=[25e3 25e3 25e3]/sqrt(3)  PhaseAngles_phases=[0 -120 +120]  Frequency=50  NonIdealSource=on  SpecifyImpedance=on  Resistance=0.8929  Inductance=16.58e-3  ShortCircuitLevel=1200e6  BaseVoltage=26e3  XRratio=7  BusType=PV  Pref=1020000000  Qref=0  Prefabc=[10e3, 10e3, 10e3]  Qrefabc=[0, 0, 0]  Qmin=-Inf  Qmax=Inf
  Source 3 960MVA,26kV,50Hz1 : spsThreePhaseSourceLib/Three-Phase Source  InternalConnection=Yg  VoltagePhases=off  Voltage=(26000)*1.27823  PhaseAngle=46.709  Voltage_phases=[25e3 25e3 25e3]/sqrt(3)  PhaseAngles_phases=[0 -120 +120]  Frequency=50  NonIdealSource=on  SpecifyImpedance=on  Resistance=0.8929  Inductance=16.58e-3  ShortCircuitLevel=960e6  BaseVoltage=26e3  XRratio=7  BusType=PV  Pref=800000000  Qref=0  Prefabc=[10e3, 10e3, 10e3]  Qrefabc=[0, 0, 0]  Qmin=-Inf  Qmax=Inf
  Subsystem_1 : Subsystem
  Subsystem_10 : Subsystem
  Subsystem_11 : Subsystem
  Subsystem_12 : Subsystem
  Subsystem_2 : Subsystem
  Subsystem_3 : Subsystem
  Subsystem_4 : Subsystem
  Subsystem_5 : Subsystem
  Subsystem_6 : Subsystem
  Subsystem_7 : Subsystem
  Subsystem_8 : Subsystem
  Subsystem_9 : Subsystem
  Subtract : Sum  Commented=on  Inputs=+-
  Subtract1 : Sum  Commented=on  Inputs=+-
  Three-Phase Breaker10 : spsThreePhaseBreakerLib/Three-Phase Breaker  InitialState=closed  SwitchA=on  SwitchB=on  SwitchC=on  SwitchTimes=[500 501]  External=off  BreakerResistance=0.01  SnubberResistance=inf  SnubberCapacitance=inf  Measurements=None
  Three-Phase Breaker12 : spsThreePhaseBreakerLib/Three-Phase Breaker  InitialState=closed  SwitchA=on  SwitchB=on  SwitchC=on  SwitchTimes=[500 501]  External=off  BreakerResistance=0.01  SnubberResistance=inf  SnubberCapacitance=inf  Measurements=None
  Three-Phase Breaker13 : spsThreePhaseBreakerLib/Three-Phase Breaker  InitialState=closed  SwitchA=on  SwitchB=on  SwitchC=on  SwitchTimes=[500 501]  External=off  BreakerResistance=0.01  SnubberResistance=inf  SnubberCapacitance=inf  Measurements=None
  Three-Phase Breaker{4..7} (4 alike) : spsThreePhaseBreakerLib/Three-Phase Breaker  InitialState=closed  SwitchA=on  SwitchB=on  SwitchC=on  SwitchTimes=[500 501]  External=off  BreakerResistance=0.01  SnubberResistance=10e6  SnubberCapacitance=inf  Measurements=None
  Three-Phase Breaker8 : spsThreePhaseBreakerLib/Three-Phase Breaker  InitialState=closed  SwitchA=on  SwitchB=on  SwitchC=on  SwitchTimes=0.7  External=off  BreakerResistance=0.01  SnubberResistance=10e6  SnubberCapacitance=inf  Measurements=None
  Three-Phase Breaker9 : spsThreePhaseBreakerLib/Three-Phase Breaker  InitialState=closed  SwitchA=on  SwitchB=on  SwitchC=on  SwitchTimes=0.7  External=off  BreakerResistance=0.01  SnubberResistance=10e6  SnubberCapacitance=inf  Measurements=None
  Three-Phase Fault1 : spsThreePhaseFaultLib/Three-Phase Fault  InitialStates=0  FaultA=on  FaultB=on  FaultC=on  GroundFault=off  SwitchTimes=[0.5 0.5+(10/50)]  External=off  SwitchStatus=NaN  FaultResistance=0.001  GroundResistance=0.01  SnubberResistance=inf  SnubberCapacitance=inf  Measurements=None
  Xmer_1 800 MVA 24 kV /400 kV : spsThreePhaseTransformerTwoWindingsLib/Three-Phase Transformer (Two Windings)  Winding1Connection=Delta (D1)  Winding2Connection=Yg  CoreType=Three single-phase transformers  SetSaturation=off  Hysteresis=off  DataFile='hysteresis'  SetInitialFlux=off  Measurements=None  UNITS=pu  NominalPower=[ 800e6 50 ]  Winding1="[ 24e3 1e-6  0]"  Winding2=[ 400e3 1e-6 0.15]  Rm=500  Lm=500  L0=0.5  Saturation="[ 0,0  ;  0.005,1.2  ;  1.0,1.4 ]"  InitialFluxes=[ 0.8 , -0.8 , 0.7 ]  BreakLoop=off  DiscreteSolver=Trapezoidal iterative  DataType=off  TransfoNumber=0
  Xmer_2 1250 MVA 26 kV / 400 kV : spsThreePhaseTransformerTwoWindingsLib/Three-Phase Transformer (Two Windings)  Winding1Connection=Delta (D1)  Winding2Connection=Yg  CoreType=Three single-phase transformers  SetSaturation=off  Hysteresis=off  DataFile='hysteresis'  SetInitialFlux=off  Measurements=None  UNITS=pu  NominalPower=[ 1250e6 50 ]  Winding1="[ 26e3 1e-6  0]"  Winding2=[ 400e3 1e-6 0.15]  Rm=500  Lm=500  L0=0.5  Saturation="[ 0,0  ;  0.005,1.2  ;  1.0,1.4 ]"  InitialFluxes=[ 0.8 , -0.8 , 0.7 ]  BreakLoop=off  DiscreteSolver=Trapezoidal iterative  DataType=off  TransfoNumber=0
  Xmer_3 1000 MVA 26 kV / 400 kV : spsThreePhaseTransformerTwoWindingsLib/Three-Phase Transformer (Two Windings)  Winding1Connection=Delta (D1)  Winding2Connection=Yg  CoreType=Three single-phase transformers  SetSaturation=off  Hysteresis=off  DataFile='hysteresis'  SetInitialFlux=off  Measurements=None  UNITS=pu  NominalPower=[1000e6 50 ]  Winding1="[ 26e3 1e-6  0]"  Winding2=[ 400e3 1e-6 0.15]  Rm=500  Lm=500  L0=0.5  Saturation="[ 0,0  ;  0.005,1.2  ;  1.0,1.4 ]"  InitialFluxes=[ 0.8 , -0.8 , 0.7 ]  BreakLoop=off  DiscreteSolver=Trapezoidal iterative  DataType=off  TransfoNumber=0
  powergui : spspowerguiLib/powergui  Priority=2  SimulationMode=Discrete  SampleTime=20e-6  frequency=60  Iterations=50  frequencyindice=50  Pbase=100e6  ErrMax=0.0001  UnitsV=kV  UnitsW=MW  buscounter=0  FunctionMessages=off  echomessages=off  EnableUseOfTLC=off  CurrentSourceSwitches=off  DisableSnubberDevices=off  DisableRonSwitches=off  DisableVfSwitches=off  DisplayEquations=off  AutomaticDiscreteSolvers=off  SolverType=Tustin  Interpol=off  ExternalGateDelay=off  methode=off  Ts=100  x0status=blocks  SPID=on  SwTol=0  HookPort=off  NonlinearTolerance=1e-4  nMaxIteration=100  ContinueOnMaxIteration=off  RestoreLinks=warning  ResistiveCurrentMeasurement=off  Frange=logspace(0,3,50)  Ylog=off  Xlog=off  ShowGrid=off  save=off  variable=ZData  structure=0  ZoomFFT=on  StartTime=0.0  cycles=2  DisplayStyle=off  fundamental=60  FreqAxis=off  MaxFrequency=1000  frequencyindicesteady=1  RmsSteady=1  display=off
  tag scope: PSS=global
  wires:
  Subtract1/1 -> Gain/1
  Subtract/1 -> Gain1/1
  Gain/1 -> Rotor Angle Deviations/1
  Gain1/1 -> Rotor Angle Deviations/2
  Gain2/1 -> Scope1/1
  Gain3/1 -> Scope1/2
  Gain4/1 -> Scope1/3
  From/1 -> Gain3/1, Subtract1/1
  From2/1 -> Gain4/1, Subtract/1
  From1/1 -> Gain2/1, Subtract1/2, Subtract/2
  Constant/1 -> [PSS]
  [Vabc_Ln_54] -> Scope/1
  [Iabc_Ln_54] -> Scope/2
  [Vabc_Ln_75] -> Demux2/1
  Demux2/1 -> Scope2/1
  [Iabc_Ln_75] -> Demux3/1
  Demux3/1 -> Scope2/2
  [Vabc_Ln_54] -> Subsystem_10/1(In1)
  [Iabc_Ln_54] -> Subsystem_10/2(In2)
  [Vabc_Ln_45] -> Subsystem_2/1(In1)
  [Iabc_Ln_45] -> Subsystem_2/2(In2)
  [Iabc_Ln_46] -> Subsystem_3/2(In2)
  [Vabc_Ln_46] -> Subsystem_3/1(In1)
  [Vabc_Ln_64] -> Subsystem_4/1(In1)
  [Iabc_Ln_64] -> Subsystem_4/2(In2)
  [Iabc_Ln_69] -> Subsystem_5/2(In2)
  [Vabc_Ln_69] -> Subsystem_5/1(In1)
  [Vabc_Ln_96] -> Subsystem_6/1(In1)
  [Iabc_Ln_96] -> Subsystem_6/2(In2)
  [Iabc_Ln_57] -> Subsystem_1/2(In2)
  [Vabc_Ln_57] -> Subsystem_1/1(In1)
  [Iabc_Ln_75] -> Subsystem_7/2(In2)
  [Vabc_Ln_75] -> Subsystem_7/1(In1)
  [Vabc_Ln_78] -> Subsystem_11/1(In1)
  [Iabc_Ln_78] -> Subsystem_11/2(In2)
  [Iabc_Ln_87] -> Subsystem_12/2(In2)
  [Vabc_Ln_87] -> Subsystem_12/1(In1)
  [Iabc_Ln_89] -> Subsystem_8/2(In2)
  [Vabc_Ln_89] -> Subsystem_8/1(In1)
  [Iabc_Ln_98] -> Subsystem_9/2(In2)
  [Vabc_Ln_98] -> Subsystem_9/1(In1)
  connections:
  B2/RConn2 -- Snb_G2/LConn2 -- Xmer_2 1250 MVA 26 kV / 400 kV/LConn2
  B2/RConn3 -- Snb_G2/LConn3 -- Xmer_2 1250 MVA 26 kV / 400 kV/LConn3
  B2/RConn1 -- Snb_G2/LConn1 -- Load Flow Bus3/LConn1 -- Xmer_2 1250 MVA 26 kV / 400 kV/LConn1
  Xmer_3 1000 MVA 26 kV / 400 kV/LConn3 -- Snb_G3/LConn3 -- B3/RConn3
  Xmer_3 1000 MVA 26 kV / 400 kV/LConn2 -- B3/RConn2 -- Snb_G3/LConn2
  Xmer_3 1000 MVA 26 kV / 400 kV/LConn1 -- B3/RConn1 -- Load Flow Bus7/LConn1 -- Snb_G3/LConn1
  B7/LConn2 -- Xmer_2 1250 MVA 26 kV / 400 kV/RConn2
  B7/LConn3 -- Xmer_2 1250 MVA 26 kV / 400 kV/RConn3
  Source 2 1200MVA,26kV,50Hz/RConn1 -- B2/LConn1
  Source 2 1200MVA,26kV,50Hz/RConn2 -- B2/LConn2
  Source 2 1200MVA,26kV,50Hz/RConn3 -- B2/LConn3
  B7/LConn1 -- Xmer_2 1250 MVA 26 kV / 400 kV/RConn1
  Line_78_b/LConn1 -- Line_78_a/RConn1
  Line_78_b/LConn2 -- Line_78_a/RConn2
  Line_78_b/LConn3 -- Line_78_a/RConn3
  B9/LConn2 -- Xmer_3 1000 MVA 26 kV / 400 kV/RConn2
  B9/LConn1 -- Xmer_3 1000 MVA 26 kV / 400 kV/RConn1
  B9/LConn3 -- Xmer_3 1000 MVA 26 kV / 400 kV/RConn3
  B_78/LConn1 -- Ln_78/RConn1
  B_78/LConn2 -- Ln_78/RConn2
  B_78/LConn3 -- Ln_78/RConn3
  B_78/RConn1 -- Line_78_a/LConn1
  B_78/RConn2 -- Line_78_a/LConn2
  B_78/RConn3 -- Line_78_a/LConn3
  Line_78_b/RConn1 -- B_87/RConn1
  Line_78_b/RConn2 -- B_87/RConn2
  Line_78_b/RConn3 -- B_87/RConn3
  Ln_87/RConn1 -- B_87/LConn1
  Ln_87/RConn2 -- B_87/LConn2
  Ln_87/RConn3 -- B_87/LConn3
  Ln_78/LConn1 -- Ln_75/LConn1 -- Load Flow Bus4/LConn1 -- B7/RConn1
  Ln_78/LConn2 -- Ln_75/LConn2 -- B7/RConn2
  Ln_78/LConn3 -- Ln_75/LConn3 -- B7/RConn3
  Line_89_b/LConn1 -- Line_89_a/RConn1
  Three-Phase Breaker4/RConn2 -- Line_89_a/LConn2
  Line_89_b/LConn2 -- Line_89_a/RConn2
  Three-Phase Breaker4/RConn1 -- Line_89_a/LConn1
  Line_89_b/RConn1 -- Three-Phase Breaker5/RConn1
  Line_89_b/LConn3 -- Line_89_a/RConn3
  Three-Phase Breaker4/LConn1 -- Ln_89/RConn1
  Ln_98/RConn1 -- Three-Phase Breaker5/LConn1
  Three-Phase Breaker4/LConn2 -- Ln_89/RConn2
  Three-Phase Breaker4/LConn3 -- Ln_89/RConn3
  Line_89_b/RConn3 -- Three-Phase Breaker5/RConn3
  Ln_98/RConn2 -- Three-Phase Breaker5/LConn2
  Line_89_b/RConn2 -- Three-Phase Breaker5/RConn2
  Three-Phase Breaker4/RConn3 -- Line_89_a/LConn3
  Ln_98/RConn3 -- Three-Phase Breaker5/LConn3
  Ln_87/LConn1 -- B8/LConn1 -- Load Flow Bus5/LConn1 -- Shunt Compensation 400 MVAr/LConn1 -- Ln_89/LConn1
  Ln_87/LConn2 -- Shunt Compensation 400 MVAr/LConn2 -- Ln_89/LConn2 -- B8/LConn2
  Ln_87/LConn3 -- Shunt Compensation 400 MVAr/LConn3 -- B8/LConn3 -- Ln_89/LConn3
  Ln_98/LConn1 -- B9/RConn1 -- Load Flow Bus6/LConn1 -- Ln_96/LConn1
  Ln_98/LConn2 -- B9/RConn2 -- Ln_96/LConn2
  Ln_98/LConn3 -- Ln_96/LConn3 -- B9/RConn3
  B8/RConn1 -- "Load A 1020 MW, 320 MVAR"/LConn1
  B8/RConn2 -- "Load A 1020 MW, 320 MVAR"/LConn2
  B8/RConn3 -- "Load A 1020 MW, 320 MVAR"/LConn3
  B6/RConn3 -- "Load C 360 MW, 120 MVAR"/LConn3
  B6/RConn2 -- "Load C 360 MW, 120 MVAR"/LConn2
  B6/RConn1 -- "Load C 360 MW, 120 MVAR"/LConn1
  B5/RConn1 -- "Load B 850 MW, 250 MVAR"/LConn1
  B5/RConn2 -- "Load B 850 MW, 250 MVAR"/LConn2
  B5/RConn3 -- "Load B 850 MW, 250 MVAR"/LConn3
  Line_69_b/LConn1 -- Line_69_a/RConn1
  Three-Phase Breaker6/RConn2 -- Line_69_a/LConn2
  Line_69_b/LConn2 -- Line_69_a/RConn2
  Three-Phase Breaker6/RConn1 -- Line_69_a/LConn1
  Line_69_b/RConn1 -- Three-Phase Breaker7/RConn1
  Line_69_b/LConn3 -- Line_69_a/RConn3
  Three-Phase Breaker6/LConn1 -- Ln_69/RConn1
  Ln_96/RConn1 -- Three-Phase Breaker7/LConn1
  Three-Phase Breaker6/LConn2 -- Ln_69/RConn2
  Three-Phase Breaker6/LConn3 -- Ln_69/RConn3
  Line_69_b/RConn3 -- Three-Phase Breaker7/RConn3
  Ln_96/RConn2 -- Three-Phase Breaker7/LConn2
  Line_69_b/RConn2 -- Three-Phase Breaker7/RConn2
  Three-Phase Breaker6/RConn3 -- Line_69_a/LConn3
  Ln_96/RConn3 -- Three-Phase Breaker7/LConn3
  Ln_64/RConn3 -- Three-Phase Breaker9/LConn3
  Three-Phase Breaker8/RConn3 -- Line_46_a/LConn3
  Line_46_b/RConn2 -- Three-Phase Breaker9/RConn2
  Ln_64/RConn2 -- Three-Phase Breaker9/LConn2
  Three-Phase Breaker8/LConn2 -- Ln_46/RConn2
  Ln_64/RConn1 -- Three-Phase Breaker9/LConn1
  Line_46_b/LConn2 -- Three-Phase Fault1/LConn2 -- Line_46_a/RConn2
  Line_46_b/RConn3 -- Three-Phase Breaker9/RConn3
  Line_46_b/RConn1 -- Three-Phase Breaker9/RConn1
  Line_46_b/LConn3 -- Three-Phase Fault1/LConn3 -- Line_46_a/RConn3
  Three-Phase Breaker8/RConn2 -- Line_46_a/LConn2
  Three-Phase Breaker8/RConn1 -- Line_46_a/LConn1
  Three-Phase Breaker8/LConn1 -- Ln_46/RConn1
  Line_46_b/LConn1 -- Line_46_a/RConn1 -- Three-Phase Fault1/LConn1
  Three-Phase Breaker8/LConn3 -- Ln_46/RConn3
  Ln_69/LConn1 -- Shunt Compensation 200 MVAr/LConn1 -- B6/LConn1 -- Ln_64/LConn1 -- Load Flow Bus8/LConn1
  Ln_69/LConn2 -- Shunt Compensation 200 MVAr/LConn2 -- B6/LConn2 -- Ln_64/LConn2
  Ln_69/LConn3 -- B6/LConn3 -- Shunt Compensation 200 MVAr/LConn3 -- Ln_64/LConn3
  Ln_57/LConn1 -- B5/LConn1 -- Ln_54/LConn1 -- Shunt Compensation 350 MVAr/LConn1 -- Load Flow Bus2/LConn1
  Ln_57/LConn2 -- Shunt Compensation 350 MVAr/LConn2 -- B5/LConn2 -- Ln_54/LConn2
  Ln_57/LConn3 -- Shunt Compensation 350 MVAr/LConn3 -- B5/LConn3 -- Ln_54/LConn3
  Three-Phase Breaker12/LConn3 -- Ln_45/RConn3
  Line_45_b/LConn1 -- Line_45_a/RConn1
  Three-Phase Breaker12/RConn1 -- Line_45_a/LConn1
  Three-Phase Breaker12/LConn1 -- Ln_45/RConn1
  Line_45_b/LConn3 -- Line_45_a/RConn3
  Line_45_b/RConn1 -- Three-Phase Breaker13/RConn1
  Line_45_b/LConn2 -- Line_45_a/RConn2
  Ln_54/RConn1 -- Three-Phase Breaker13/LConn1
  Ln_54/RConn2 -- Three-Phase Breaker13/LConn2
  Line_45_b/RConn2 -- Three-Phase Breaker13/RConn2
  Three-Phase Breaker12/RConn3 -- Line_45_a/LConn3
  Ln_54/RConn3 -- Three-Phase Breaker13/LConn3
  Ln_75/RConn3 -- B_75/LConn3
  Three-Phase Breaker10/RConn3 -- Line_57_a/LConn3
  Line_57_b/RConn2 -- B_75/RConn2
  Ln_75/RConn2 -- B_75/LConn2
  Three-Phase Breaker12/LConn2 -- Ln_45/RConn2
  Line_45_b/RConn3 -- Three-Phase Breaker13/RConn3
  Three-Phase Breaker10/LConn2 -- Ln_57/RConn2
  Ln_75/RConn1 -- B_75/LConn1
  Three-Phase Breaker10/LConn1 -- Ln_57/RConn1
  Line_57_b/LConn2 -- Line_57_a/RConn2
  Line_57_b/RConn3 -- B_75/RConn3
  Line_57_b/RConn1 -- B_75/RConn1
  Line_57_b/LConn3 -- Line_57_a/RConn3
  Three-Phase Breaker10/RConn2 -- Line_57_a/LConn2
  Three-Phase Breaker10/RConn1 -- Line_57_a/LConn1
  Line_57_b/LConn1 -- Line_57_a/RConn1
  Three-Phase Breaker10/LConn3 -- Ln_57/RConn3
  Three-Phase Breaker12/RConn2 -- Line_45_a/LConn2
  Xmer_1 800 MVA 24 kV /400 kV/RConn1 -- B4/LConn1
  Xmer_1 800 MVA 24 kV /400 kV/RConn2 -- B4/LConn2
  Xmer_1 800 MVA 24 kV /400 kV/RConn3 -- B4/LConn3
  B1/RConn1 -- Load Flow Bus/LConn1 -- Snb_G1/LConn1 -- Xmer_1 800 MVA 24 kV /400 kV/LConn1
  B1/RConn2 -- Snb_G1/LConn2 -- Xmer_1 800 MVA 24 kV /400 kV/LConn2
  B1/RConn3 -- Snb_G1/LConn3 -- Xmer_1 800 MVA 24 kV /400 kV/LConn3
  Ln_45/LConn1 -- Load Flow Bus1/LConn1 -- B4/RConn1 -- Ln_46/LConn1
  Ln_45/LConn2 -- Ln_46/LConn2 -- B4/RConn2
  Ln_45/LConn3 -- Ln_46/LConn3 -- B4/RConn3
  Source 3 960MVA,26kV,50Hz1/RConn1 -- B3/LConn1
  Source 3 960MVA,26kV,50Hz1/RConn2 -- B3/LConn2
  Source 3 960MVA,26kV,50Hz1/RConn3 -- B3/LConn3
  Source 1 776.5MVA,24kV,50Hz1/RConn1 -- B1/LConn1
  Source 1 776.5MVA,24kV,50Hz1/RConn2 -- B1/LConn2
  Source 1 776.5MVA,24kV,50Hz1/RConn3 -- B1/LConn3
